simulink model "ElevatorPlant_Storage_A"  (R2015b)
(part 3 of 8)

      state Updating_button_0
        en:
        BUTTON=MAX_BUT;
      state Updating_button_1
        en:
        BUTTON=MIN_BUT;
      (junction 29277) -> Button_detection.Max_Min_assignment.Min_but [order 1] : [(MAX_BUT-FLOOR)>(FLOOR-MIN_BUT)]
      Button_detection.Max_Min_assignment.Min_but -> (junction 29278)
      (junction 29279) -> (junction 29277) [order 1] : [not(FLAG_STOP) && MOTION==2 && FLAG==3]
      (default) -> (junction 29279)
      (junction 29277) -> (junction 29280) [order 2]
      (junction 29278) -> (junction 29281)
      (junction 29279) -> (junction 29282) [order 2]
      (junction 29280) -> Button_detection.Max_Min_assignment.Max_but [order 1] : [(MAX_BUT-FLOOR)<(FLOOR-MIN_BUT)]
      Button_detection.Max_Min_assignment.Max_but -> (junction 29281)
      (junction 29280) -> Button_detection.Max_Min_assignment.First_but [order 2]
      (junction 29281) -> (junction 29284)
      Button_detection.Max_Min_assignment.First_but -> (junction 29283)
      (junction 29283) -> (junction 29282)
      (junction 29284) -> (junction 29283)
      (junction 29282) -> (junction 29285)
      (junction 29286) -> (junction 29287) [order 1] : [MOTION==0]
          | {MOTION=1;
          | UPDATE=true;}
      (junction 29287) -> Button_detection.Max_Min_assignment.Max_but1 [order 1] : [BUTTON_UP(2)]
      Button_detection.Max_Min_assignment.Max_but1 -> (junction 29288)
      (junction 29285) -> (junction 29286) [order 1] : [BUTTON==FLOOR && EXTEND]
          | {EXTEND=false;}
      (junction 29285) -> (junction 29299) [order 2]
      (junction 29286) -> (junction 29291) [order 2]
      (junction 29287) -> (junction 29289) [order 2]
      (junction 29288) -> (junction 29290)
      (junction 29289) -> Button_detection.Max_Min_assignment.Max_but2 [order 1] : [BUTTON_UP(1)]
      Button_detection.Max_Min_assignment.Max_but2 -> (junction 29290)
      (junction 29289) -> Button_detection.Max_Min_assignment.Max_but3 [order 2]
      (junction 29290) -> (junction 29293)
      Button_detection.Max_Min_assignment.Max_but3 -> (junction 29292)
      (junction 29292) -> (junction 29291)
      (junction 29293) -> (junction 29292)
      (junction 29291) -> (junction 29294)
      (junction 29294) -> (junction 29295) [order 1] : [MOTION==1]
          | {MOTION=0;
          | UPDATE=true;}
      (junction 29295) -> Button_detection.Max_Min_assignment.Min_but1 [order 1] : [BUTTON_DOWN(1)]
      Button_detection.Max_Min_assignment.Min_but1 -> (junction 29296)
      (junction 29294) -> (junction 29300) [order 2]
      (junction 29295) -> (junction 29297) [order 2]
      (junction 29296) -> (junction 29298)
      (junction 29297) -> Button_detection.Max_Min_assignment.Min_but2 [order 1] : [BUTTON_DOWN(2)]
      Button_detection.Max_Min_assignment.Min_but2 -> (junction 29298)
      (junction 29297) -> Button_detection.Max_Min_assignment.Min_but3 [order 2]
      (junction 29298) -> (junction 29302)
      Button_detection.Max_Min_assignment.Min_but3 -> (junction 29301)
      (junction 29300) -> (junction 29299)
      (junction 29301) -> (junction 29300)
      (junction 29302) -> (junction 29301)
      (junction 29299) -> (junction 29304)
      Button_detection.Max_Min_assignment.MAX -> (junction 29303)
      (junction 29304) -> (junction 29305) [order 1] : [PUSHED]
      (junction 29305) -> (junction 29306) [order 1] : [not(BUT_TEMP==FLOOR) || not(MOTION==2)]
      (junction 29306) -> Button_detection.Max_Min_assignment.MAX [order 1] : [MAX_BUT<BUT_TEMP && not(UPDATE)]
      (junction 29303) -> (junction 29308)
      (junction 29304) -> (junction 29318) [order 2]
      (junction 29305) -> (junction 29311) [order 2]
      (junction 29306) -> (junction 29307) [order 2]
      (junction 29308) -> (junction 29307)
      (junction 29307) -> (junction 29309)
      (junction 29309) -> Button_detection.Max_Min_assignment.MIN [order 1] : [MIN_BUT>BUT_TEMP && not(UPDATE)]
      Button_detection.Max_Min_assignment.MIN -> (junction 29310)
      (junction 29309) -> (junction 29312) [order 2]
      (junction 29310) -> (junction 29313)
      (junction 29312) -> (junction 29311)
      (junction 29313) -> (junction 29312)
      (junction 29311) -> (junction 29314)
      (junction 29314) -> Button_detection.Max_Min_assignment.Updating_button_0 [order 1] : [MOTION==0]
      Button_detection.Max_Min_assignment.Updating_button_0 -> (junction 29315)
      (junction 29314) -> (junction 29316) [order 2]
      (junction 29315) -> (junction 29317)
      (junction 29316) -> Button_detection.Max_Min_assignment.Updating_button_1 [order 1] : [MOTION==1]
      Button_detection.Max_Min_assignment.Updating_button_1 -> (junction 29317)
      (junction 29316) -> (junction 29319) [order 2]
      (junction 29317) -> (junction 29320)
      (junction 29319) -> (junction 29318)
      (junction 29320) -> (junction 29319)
    state GoTo_PositionControl
      en:
      BUTTON=BUT_TEMP;
      FLAG=2;
    state Emergency
      en:
      FLAG_EMG=true;
      FLAG=4;
    state Timer_EME
      state Set_tmr
        en:
        Q_EME=true;
      state Counting
        en:
        ET_EME= ET_EME + 1;
        Q_EME=false;
      state Set
        en:
        IN_EME=true;
        PT_EME=3;
      (junction 29410) -> Button_detection.Timer_EME.Set_tmr [order 1] : [ET_EME==PT_EME]
      Button_detection.Timer_EME.Set_tmr -> (junction 29411)
      Button_detection.Timer_EME.Counting -> (junction 29410)
      (junction 29410) -> (junction 29411) [order 2]
      (default) -> Button_detection.Timer_EME.Set
      Button_detection.Timer_EME.Set -> (junction 29412)
      (junction 29412) -> Button_detection.Timer_EME.Counting [order 1] : [ET_EME<PT_EME]
      (junction 29412) -> (junction 29411) [order 2]
    state Not_Emergency
      en:
      IN_EME=false;
      ET_EME=0;
    state SwitchingOFF_LEDs
      en:
      LPD3=false;
      LPD2=false;
      LPS2=false;
      LPD1=false;
      LPS1=false;
      LPS0=false;
    (default) -> (junction 29011)
    (junction 29011) -> (junction 29012) [order 1] : [FLAG==1 && not(PUSHED)]
        | {BUTTON=FLOOR;
        | BUT_TEMP=BUTTON;
        | BUT_1=FLOOR;}
    (junction 29012) -> Button_detection.Timer_LL [order 1] : [not(FLAG_STOP)]
    Button_detection.Save_energy -> (junction 29013)
    Button_detection.Timer_LL -> Button_detection.Save_energy
    (junction 29012) -> (junction 29015) [order 2]
    (junction 29011) -> (junction 29014) [order 2]
    (junction 29013) -> (junction 29016)
    (junction 29015) -> (junction 29014)
    (junction 29016) -> (junction 29015)
    (junction 29014) -> Button_detection.BUTTON_CAR
    Button_detection.BUTTON_UP -> Button_detection.BUTTON_DOWN
    Button_detection.BUTTON_DOWN -> Button_detection.Max_Min_assignment
    Button_detection.Max_Min_assignment -> (junction 29017)
    Button_detection.BUTTON_CAR -> Button_detection.BUTTON_UP
    (junction 29017) -> (junction 29019)
    (junction 29019) -> (junction 29018)
    (junction 29018) -> (junction 29021)
    Button_detection.GoTo_PositionControl -> (junction 29020)
    (junction 29021) -> (junction 29022) [order 1] : [FLAG==1]
    (junction 29022) -> Button_detection.GoTo_PositionControl [order 1] : [PUSHED]
    (junction 29020) -> (junction 29024)
    (junction 29021) -> (junction 29032) [order 2]
    (junction 29022) -> (junction 29023) [order 2]
    (junction 29024) -> (junction 29023)
    (junction 29023) -> (junction 29026)
    Button_detection.Emergency -> (junction 29025)
    (junction 29026) -> Button_detection.Timer_EME [order 1] : [STOP]
        | {IN_LL=false; ET_LL=0;FLAG=1;}
    Button_detection.Timer_EME -> (junction 29027)
    (junction 29027) -> Button_detection.Emergency [order 1] : [Q_EME]
    (junction 29025) -> (junction 29029)
    (junction 29026) -> Button_detection.Not_Emergency [order 2]
    (junction 29027) -> (junction 29028) [order 2]
    (junction 29029) -> (junction 29028)
    (junction 29028) -> (junction 29031)
    Button_detection.Not_Emergency -> (junction 29031)
    Button_detection.SwitchingOFF_LEDs -> (junction 29030)
    (junction 29031) -> Button_detection.SwitchingOFF_LEDs [order 1] : [FLAG_STOP && FLAG==2]
    (junction 29030) -> (junction 29034)
    (junction 29031) -> (junction 29033) [order 2]
    (junction 29033) -> (junction 29032)
    (junction 29034) -> (junction 29033)
  state Position_control
    state Going_UP
      en:
      SALI=true;
      MOTION=0;
      FLAG_STOP=false;
    state Button_detection
      state Save_energy
        en:
        LL=not(Q_LL);
      state Timer_LL
        state Set_tmr
          en:
          Q_LL=true;
        state Counting
          en:
          ET_LL= ET_LL + 1;
          Q_LL=false;
        state Set
          en:
          IN_LL=true;
          PT_LL=10;
        (junction 68131) -> Position_control.Button_detection.Timer_LL.Set_tmr [order 1] : [ET_LL==PT_LL]
        Position_control.Button_detection.Timer_LL.Set_tmr -> (junction 68132)
        Position_control.Button_detection.Timer_LL.Counting -> (junction 68131)
        (junction 68131) -> (junction 68132) [order 2]
        (default) -> Position_control.Button_detection.Timer_LL.Set
        Position_control.Button_detection.Timer_LL.Set -> (junction 68133)
        (junction 68133) -> Position_control.Button_detection.Timer_LL.Counting [order 1] : [ET_LL<PT_LL]
        (junction 68133) -> (junction 68132) [order 2]
      state BUTTON_DOWN
        state Button_DOWN_1
          en:
          BUTTON_DOWN(2)=true;
          BUT_TEMP=1;
          LPD1=true;
          PUSHED=true;
          UPDATE=false;
          IN_LL=false; ET_LL=0;
        state First_but_1
          en:
          BUT_1=BUT_TEMP;
          FIRST_BUT=false;
        state Button_DOWN_2
          en:
          BUTTON_DOWN(3)=true;
          BUT_TEMP=2;
          LPD2=true;
          PUSHED=true;
          UPDATE=false;
          IN_LL=false; ET_LL=0;
        state First_but_2
          en:
          BUT_1=BUT_TEMP;
          FIRST_BUT=false;
        state Button_DOWN_3
          en:
          BUTTON_DOWN(4)=true;
          BUT_TEMP=3;
          LPD3=true;
          PUSHED=true;
          UPDATE=false;
          IN_LL=false; ET_LL=0;
        state First_but_3
          en:
          BUT_1=BUT_TEMP;
          FIRST_BUT=false;
        (default) -> (junction 68146)
        (junction 68146) -> Position_control.Button_detection.BUTTON_DOWN.Button_DOWN_1 [order 1] : [PD1]
        Position_control.Button_detection.BUTTON_DOWN.Button_DOWN_1 -> (junction 68147)
        (junction 68147) -> Position_control.Button_detection.BUTTON_DOWN.First_but_1 [order 1] : [FIRST_BUT && not(RPC1)]
        Position_control.Button_detection.BUTTON_DOWN.First_but_1 -> (junction 68148)
        (junction 68146) -> (junction 68149) [order 2]
        (junction 68147) -> (junction 68150) [order 2]
        (junction 68148) -> (junction 68151)
        (junction 68150) -> (junction 68149)
        (junction 68151) -> (junction 68150)
        (junction 68149) -> (junction 68152)
        (junction 68152) -> Position_control.Button_detection.BUTTON_DOWN.Button_DOWN_2 [order 1] : [PD2]
        Position_control.Button_detection.BUTTON_DOWN.Button_DOWN_2 -> (junction 68153)
        (junction 68153) -> Position_control.Button_detection.BUTTON_DOWN.First_but_2 [order 1] : [FIRST_BUT && not(RPC2)]
        Position_control.Button_detection.BUTTON_DOWN.First_but_2 -> (junction 68154)
        (junction 68152) -> (junction 68155) [order 2]
        (junction 68153) -> (junction 68156) [order 2]
        (junction 68154) -> (junction 68157)
        (junction 68156) -> (junction 68155)
        (junction 68157) -> (junction 68156)
        (junction 68155) -> (junction 68158)
        (junction 68158) -> Position_control.Button_detection.BUTTON_DOWN.Button_DOWN_3 [order 1] : [PD3]
        Position_control.Button_detection.BUTTON_DOWN.Button_DOWN_3 -> (junction 68159)
        (junction 68159) -> Position_control.Button_detection.BUTTON_DOWN.First_but_3 [order 1] : [FIRST_BUT && not(RPC3)]
        Position_control.Button_detection.BUTTON_DOWN.First_but_3 -> (junction 68160)
        (junction 68158) -> (junction 68161) [order 2]
        (junction 68159) -> (junction 68162) [order 2]
        (junction 68160) -> (junction 68163)
        (junction 68162) -> (junction 68161)
        (junction 68163) -> (junction 68162)
      state BUTTON_CAR
        state Button_CAR_0
          en:
          BUTTON_CAR(1)=true;
          BUT_TEMP=0;
          LPC0=true;
          PUSHED=true;
          UPDATE=false;
          IN_LL=false; ET_LL=0;
        state First_but_0
          en:
          BUT_1=BUT_TEMP;
          FIRST_BUT=false;
        state Button_CAR_1
          en:
          BUTTON_CAR(2)=true;
          BUT_TEMP=1;
          LPC1=true;
          PUSHED=true;
          UPDATE=false;
          IN_LL=false; ET_LL=0;
        state First_but_1
          en:
          BUT_1=BUT_TEMP;
          FIRST_BUT=false;
        state Button_CAR_2
          en:
          BUTTON_CAR(3)=true;
          BUT_TEMP=2;
          LPC2=true;
          PUSHED=true;
          UPDATE=false;
          IN_LL=false; ET_LL=0;
        state First_but_2
          en:
          BUT_1=BUT_TEMP;
          FIRST_BUT=false;
        state Button_CAR_3
          en:
          BUTTON_CAR(4)=true;
          BUT_TEMP=3;
          LPC3=true;
          PUSHED=true;
          UPDATE=false;
          IN_LL=false; ET_LL=0;
        state First_but_3
          en:
          BUT_1=BUT_TEMP;
          FIRST_BUT=false;
        (default) -> (junction 68201)
        (junction 68201) -> Position_control.Button_detection.BUTTON_CAR.Button_CAR_0 [order 1] : [P0]
        Position_control.Button_detection.BUTTON_CAR.Button_CAR_0 -> (junction 68202)
        (junction 68202) -> Position_control.Button_detection.BUTTON_CAR.First_but_0 [order 1] : [FIRST_BUT && not(RPC0)]
        Position_control.Button_detection.BUTTON_CAR.First_but_0 -> (junction 68203)
        (junction 68201) -> (junction 68204) [order 2]
        (junction 68202) -> (junction 68205) [order 2]
        (junction 68203) -> (junction 68206)
        (junction 68205) -> (junction 68204)
        (junction 68206) -> (junction 68205)
        (junction 68204) -> (junction 68209)
        Position_control.Button_detection.BUTTON_CAR.Button_CAR_1 -> (junction 68207)
        (junction 68207) -> Position_control.Button_detection.BUTTON_CAR.First_but_1 [order 1] : [FIRST_BUT && not(RPC1)]
        Position_control.Button_detection.BUTTON_CAR.First_but_1 -> (junction 68208)
        (junction 68207) -> (junction 68211) [order 2]
        (junction 68208) -> (junction 68212)
        (junction 68209) -> Position_control.Button_detection.BUTTON_CAR.Button_CAR_1 [order 1] : [P1]
        (junction 68209) -> (junction 68210) [order 2]
        (junction 68211) -> (junction 68210)
        (junction 68212) -> (junction 68211)
        (junction 68210) -> (junction 68213)
        (junction 68213) -> Position_control.Button_detection.BUTTON_CAR.Button_CAR_2 [order 1] : [P2]
        Position_control.Button_detection.BUTTON_CAR.Button_CAR_2 -> (junction 68214)
        (junction 68214) -> Position_control.Button_detection.BUTTON_CAR.First_but_2 [order 1] : [FIRST_BUT && not(RPC2)]
        Position_control.Button_detection.BUTTON_CAR.First_but_2 -> (junction 68215)
        (junction 68213) -> (junction 68216) [order 2]
        (junction 68214) -> (junction 68217) [order 2]
        (junction 68215) -> (junction 68218)
        (junction 68217) -> (junction 68216)
        (junction 68218) -> (junction 68217)
        (junction 68216) -> (junction 68219)
        (junction 68219) -> Position_control.Button_detection.BUTTON_CAR.Button_CAR_3 [order 1] : [P3]
        Position_control.Button_detection.BUTTON_CAR.Button_CAR_3 -> (junction 68220)
        (junction 68220) -> Position_control.Button_detection.BUTTON_CAR.First_but_3 [order 1] : [FIRST_BUT && not(RPC3)]
        Position_control.Button_detection.BUTTON_CAR.First_but_3 -> (junction 68221)
        (junction 68219) -> (junction 68222) [order 2]
        (junction 68220) -> (junction 68223) [order 2]
        (junction 68221) -> (junction 68224)
        (junction 68223) -> (junction 68222)
        (junction 68224) -> (junction 68223)
      state BUTTON_UP
        state Button_UP_0
          en:
          BUTTON_UP(1)=true;
          BUT_TEMP=0;
          LPS0=true;
          PUSHED=true;
          UPDATE=false;
          IN_LL=false; ET_LL=0;
        state First_but_0
          en:
          BUT_1=BUT_TEMP;
          FIRST_BUT=false;
        state Button_UP_1
          en:
          BUTTON_UP(2)=true;
          BUT_TEMP=1;
          LPS1=true;
          PUSHED=true;
          UPDATE=false;
          IN_LL=false; ET_LL=0;
        state First_but_1
          en:
          BUT_1=BUT_TEMP;
          FIRST_BUT=false;
        state Button_UP_2
          en:
          BUTTON_UP(3)=true;
          BUT_TEMP=2;
          LPS2=true;
          PUSHED=true;
          UPDATE=false;
          IN_LL=false; ET_LL=0;
        state First_but_2
          en:
          BUT_1=BUT_TEMP;
          FIRST_BUT=false;
        (junction 68274) -> Position_control.Button_detection.BUTTON_UP.Button_UP_0 [order 1] : [PS0]
        Position_control.Button_detection.BUTTON_UP.Button_UP_0 -> (junction 68275)
        (junction 68275) -> Position_control.Button_detection.BUTTON_UP.First_but_0 [order 1] : [FIRST_BUT && not(RPC0)]
        Position_control.Button_detection.BUTTON_UP.First_but_0 -> (junction 68276)
        (default) -> (junction 68274)
        (junction 68274) -> (junction 68279) [order 2]
        (junction 68275) -> (junction 68277) [order 2]
        (junction 68276) -> (junction 68278)
        (junction 68278) -> (junction 68277)
        (junction 68277) -> (junction 68279)
        (junction 68279) -> (junction 68280)
        (junction 68280) -> Position_control.Button_detection.BUTTON_UP.Button_UP_1 [order 1] : [PS1]
        Position_control.Button_detection.BUTTON_UP.Button_UP_1 -> (junction 68281)
        (junction 68281) -> Position_control.Button_detection.BUTTON_UP.First_but_1 [order 1] : [FIRST_BUT && not(RPC1)]
        Position_control.Button_detection.BUTTON_UP.First_but_1 -> (junction 68282)
        (junction 68280) -> (junction 68283) [order 2]
        (junction 68281) -> (junction 68284) [order 2]
        (junction 68282) -> (junction 68285)
        (junction 68284) -> (junction 68283)
        (junction 68285) -> (junction 68284)
        (junction 68283) -> (junction 68287)
        Position_control.Button_detection.BUTTON_UP.First_but_2 -> (junction 68286)
        (junction 68286) -> (junction 68291)
        (junction 68287) -> Position_control.Button_detection.BUTTON_UP.Button_UP_2 [order 1] : [PS2]
        Position_control.Button_detection.BUTTON_UP.Button_UP_2 -> (junction 68288)
        (junction 68288) -> Position_control.Button_detection.BUTTON_UP.First_but_2 [order 1] : [FIRST_BUT && not(RPC2)]
        (junction 68287) -> (junction 68289) [order 2]
        (junction 68288) -> (junction 68290) [order 2]
        (junction 68290) -> (junction 68289)
        (junction 68291) -> (junction 68290)
      state Max_Min_assignment
        state Min_but
          en:
          BUTTON=MIN_BUT;
        state Max_but
          en:
          BUTTON=MAX_BUT;
        state First_but
          en:
          BUTTON=BUT_1;
        state Max_but1
          en:
          MAX_BUT=2;
        state Max_but2
          en:
          MAX_BUT=1;
        state Max_but3
          en:
          MAX_BUT=0;
        state Min_but1
          en:
          MIN_BUT=1;
        state Min_but2
          en:
          MIN_BUT=2;
        state Min_but3
          en:
          MIN_BUT=3;
        state MAX
          en:
          MAX_BUT=BUT_TEMP;
        state MIN
          en:
          MIN_BUT=BUT_TEMP;
        state Updating_button_0
          en:
          BUTTON=MAX_BUT;
        state Updating_button_1
          en:
          BUTTON=MIN_BUT;
        (junction 68329) -> Position_control.Button_detection.Max_Min_assignment.Min_but [order 1] : [(MAX_BUT-FLOOR)>(FLOOR-MIN_BUT)]
        Position_control.Button_detection.Max_Min_assignment.Min_but -> (junction 68330)
        (junction 68331) -> (junction 68329) [order 1] : [not(FLAG_STOP) && MOTION==2 && FLAG==3]
        (default) -> (junction 68331)
        (junction 68329) -> (junction 68332) [order 2]
        (junction 68330) -> (junction 68333)
        (junction 68331) -> (junction 68334) [order 2]
        (junction 68332) -> Position_control.Button_detection.Max_Min_assignment.Max_but [order 1] : [(MAX_BUT-FLOOR)<(FLOOR-MIN_BUT)]
        Position_control.Button_detection.Max_Min_assignment.Max_but -> (junction 68333)
        (junction 68332) -> Position_control.Button_detection.Max_Min_assignment.First_but [order 2]
        (junction 68333) -> (junction 68336)
        Position_control.Button_detection.Max_Min_assignment.First_but -> (junction 68335)
        (junction 68335) -> (junction 68334)
        (junction 68336) -> (junction 68335)
        (junction 68334) -> (junction 68337)
        (junction 68338) -> (junction 68339) [order 1] : [MOTION==0]
            | {MOTION=1;
            | UPDATE=true;}
        (junction 68339) -> Position_control.Button_detection.Max_Min_assignment.Max_but1 [order 1] : [BUTTON_UP(2)]
        Position_control.Button_detection.Max_Min_assignment.Max_but1 -> (junction 68340)
        (junction 68337) -> (junction 68338) [order 1] : [BUTTON==FLOOR && EXTEND]
            | {EXTEND=false;}
        (junction 68337) -> (junction 68351) [order 2]
        (junction 68338) -> (junction 68343) [order 2]
        (junction 68339) -> (junction 68341) [order 2]
        (junction 68340) -> (junction 68342)
        (junction 68341) -> Position_control.Button_detection.Max_Min_assignment.Max_but2 [order 1] : [BUTTON_UP(1)]
        Position_control.Button_detection.Max_Min_assignment.Max_but2 -> (junction 68342)
        (junction 68341) -> Position_control.Button_detection.Max_Min_assignment.Max_but3 [order 2]
        (junction 68342) -> (junction 68345)
        Position_control.Button_detection.Max_Min_assignment.Max_but3 -> (junction 68344)
        (junction 68344) -> (junction 68343)
        (junction 68345) -> (junction 68344)
        (junction 68343) -> (junction 68346)
        (junction 68346) -> (junction 68347) [order 1] : [MOTION==1]
            | {MOTION=0;
            | UPDATE=true;}
        (junction 68347) -> Position_control.Button_detection.Max_Min_assignment.Min_but1 [order 1] : [BUTTON_DOWN(1)]
        Position_control.Button_detection.Max_Min_assignment.Min_but1 -> (junction 68348)
        (junction 68346) -> (junction 68352) [order 2]
        (junction 68347) -> (junction 68349) [order 2]
        (junction 68348) -> (junction 68350)
        (junction 68349) -> Position_control.Button_detection.Max_Min_assignment.Min_but2 [order 1] : [BUTTON_DOWN(2)]
        Position_control.Button_detection.Max_Min_assignment.Min_but2 -> (junction 68350)
        (junction 68349) -> Position_control.Button_detection.Max_Min_assignment.Min_but3 [order 2]
        (junction 68350) -> (junction 68354)
        Position_control.Button_detection.Max_Min_assignment.Min_but3 -> (junction 68353)
        (junction 68352) -> (junction 68351)
        (junction 68353) -> (junction 68352)
        (junction 68354) -> (junction 68353)
        (junction 68351) -> (junction 68356)
        Position_control.Button_detection.Max_Min_assignment.MAX -> (junction 68355)
        (junction 68356) -> (junction 68357) [order 1] : [PUSHED]
        (junction 68357) -> (junction 68358) [order 1] : [not(BUT_TEMP==FLOOR) || not(MOTION==2)]
        (junction 68358) -> Position_control.Button_detection.Max_Min_assignment.MAX [order 1] : [MAX_BUT<BUT_TEMP && not(UPDATE)]
        (junction 68355) -> (junction 68360)
        (junction 68356) -> (junction 68370) [order 2]
        (junction 68357) -> (junction 68363) [order 2]
        (junction 68358) -> (junction 68359) [order 2]
        (junction 68360) -> (junction 68359)
        (junction 68359) -> (junction 68361)
        (junction 68361) -> Position_control.Button_detection.Max_Min_assignment.MIN [order 1] : [MIN_BUT>BUT_TEMP && not(UPDATE)]
        Position_control.Button_detection.Max_Min_assignment.MIN -> (junction 68362)
        (junction 68361) -> (junction 68364) [order 2]
        (junction 68362) -> (junction 68365)
        (junction 68364) -> (junction 68363)
        (junction 68365) -> (junction 68364)
        (junction 68363) -> (junction 68366)
        (junction 68366) -> Position_control.Button_detection.Max_Min_assignment.Updating_button_0 [order 1] : [MOTION==0]
        Position_control.Button_detection.Max_Min_assignment.Updating_button_0 -> (junction 68367)
        (junction 68366) -> (junction 68368) [order 2]
        (junction 68367) -> (junction 68369)
        (junction 68368) -> Position_control.Button_detection.Max_Min_assignment.Updating_button_1 [order 1] : [MOTION==1]
        Position_control.Button_detection.Max_Min_assignment.Updating_button_1 -> (junction 68369)
        (junction 68368) -> (junction 68371) [order 2]
        (junction 68369) -> (junction 68372)
        (junction 68371) -> (junction 68370)
        (junction 68372) -> (junction 68371)
      state GoTo_PositionControl
        en:
        BUTTON=BUT_TEMP;
        FLAG=2;
      state Emergency
        en:
        FLAG_EMG=true;
        FLAG=4;
      state Timer_EME
        state Set_tmr
          en:
          Q_EME=true;
        state Counting
          en:
          ET_EME= ET_EME + 1;
          Q_EME=false;
        state Set
          en:
          IN_EME=true;
          PT_EME=3;
        (junction 68462) -> Position_control.Button_detection.Timer_EME.Set_tmr [order 1] : [ET_EME==PT_EME]
        Position_control.Button_detection.Timer_EME.Set_tmr -> (junction 68463)
        Position_control.Button_detection.Timer_EME.Counting -> (junction 68462)
        (junction 68462) -> (junction 68463) [order 2]
        (default) -> Position_control.Button_detection.Timer_EME.Set
        Position_control.Button_detection.Timer_EME.Set -> (junction 68464)
        (junction 68464) -> Position_control.Button_detection.Timer_EME.Counting [order 1] : [ET_EME<PT_EME]
        (junction 68464) -> (junction 68463) [order 2]
      state Not_Emergency
        en:
        IN_EME=false;
        ET_EME=0;
      state SwitchingOFF_LEDs
        en:
        LPD3=false;
        LPD2=false;
        LPS2=false;
        LPD1=false;
        LPS1=false;
        LPS0=false;
      (default) -> (junction 68063)
      (junction 68063) -> (junction 68064) [order 1] : [FLAG==1 && not(PUSHED)]
          | {BUTTON=FLOOR;
          | BUT_TEMP=BUTTON;
          | BUT_1=FLOOR;}
      (junction 68064) -> Position_control.Button_detection.Timer_LL [order 1] : [not(FLAG_STOP)]
      Position_control.Button_detection.Save_energy -> (junction 68065)
      Position_control.Button_detection.Timer_LL -> Position_control.Button_detection.Save_energy
      (junction 68064) -> (junction 68067) [order 2]
      (junction 68063) -> (junction 68066) [order 2]
      (junction 68065) -> (junction 68068)
      (junction 68067) -> (junction 68066)
      (junction 68068) -> (junction 68067)
      (junction 68066) -> Position_control.Button_detection.BUTTON_CAR
      Position_control.Button_detection.BUTTON_UP -> Position_control.Button_detection.BUTTON_DOWN
      Position_control.Button_detection.BUTTON_DOWN -> Position_control.Button_detection.Max_Min_assignment
      Position_control.Button_detection.Max_Min_assignment -> (junction 68069)
      Position_control.Button_detection.BUTTON_CAR -> Position_control.Button_detection.BUTTON_UP
      (junction 68069) -> (junction 68071)
      (junction 68071) -> (junction 68070)
      (junction 68070) -> (junction 68073)
      Position_control.Button_detection.GoTo_PositionControl -> (junction 68072)
      (junction 68073) -> (junction 68074) [order 1] : [FLAG==1]
      (junction 68074) -> Position_control.Button_detection.GoTo_PositionControl [order 1] : [PUSHED]
      (junction 68072) -> (junction 68076)
      (junction 68073) -> (junction 68084) [order 2]
      (junction 68074) -> (junction 68075) [order 2]
      (junction 68076) -> (junction 68075)
      (junction 68075) -> (junction 68078)
      Position_control.Button_detection.Emergency -> (junction 68077)
      (junction 68078) -> Position_control.Button_detection.Timer_EME [order 1] : [STOP]
          | {IN_LL=false; ET_LL=0;FLAG=1;}
      Position_control.Button_detection.Timer_EME -> (junction 68079)
      (junction 68079) -> Position_control.Button_detection.Emergency [order 1] : [Q_EME]
      (junction 68077) -> (junction 68081)
      (junction 68078) -> Position_control.Button_detection.Not_Emergency [order 2]
      (junction 68079) -> (junction 68080) [order 2]
      (junction 68081) -> (junction 68080)
      (junction 68080) -> (junction 68083)
      Position_control.Button_detection.Not_Emergency -> (junction 68083)
      Position_control.Button_detection.SwitchingOFF_LEDs -> (junction 68082)
      (junction 68083) -> Position_control.Button_detection.SwitchingOFF_LEDs [order 1] : [FLAG_STOP && FLAG==2]
      (junction 68082) -> (junction 68086)
      (junction 68083) -> (junction 68085) [order 2]
      (junction 68085) -> (junction 68084)
      (junction 68086) -> (junction 68085)
    state INT_Stop
      state Stop
        en: SALI=false;
        FLAG=3;
      state Stop1
        en: SALI=false;
        FLAG=3;
      state Stop2
        en: SCENDI=false;
        FLAG=3;
      state Stop3
        en: SCENDI=false;
        FLAG=3;
      Position_control.INT_Stop.Stop -> (junction 29850)
      (default) -> (junction 12494)
      (junction 12494) -> (junction 12497) [order 1] : [MOTION==0]
      (junction 12497) -> (junction 12481) [order 1] : [FLOOR==1]
      (junction 12481) -> Position_control.INT_Stop.Stop [order 1] : [RPC1 && (BUTTON_CAR(2) || BUTTON_UP(2))]
      (junction 29850) -> (junction 29857)
      (junction 12494) -> (junction 29876) [order 2]
      (junction 12497) -> (junction 29848) [order 2]
      (junction 12481) -> (junction 29855) [order 2]
      (junction 29855) -> (junction 29857)
      (junction 29857) -> (junction 29852)
      (junction 12487) -> Position_control.INT_Stop.Stop1 [order 1] : [RPC2 && (BUTTON_CAR(3) || BUTTON_UP(3))]
      (junction 29848) -> (junction 12487) [order 1] : [FLOOR==2]
      Position_control.INT_Stop.Stop1 -> (junction 29852)
      (junction 29848) -> (junction 29874) [order 2]
      (junction 12487) -> (junction 29861) [order 2]
      (junction 29852) -> (junction 29862)
      (junction 29861) -> (junction 29862)
      (junction 29862) -> (junction 29866)
      (junction 29874) -> (junction 29876)
      (junction 29866) -> (junction 29874)
      (junction 29876) -> (junction 29878)
      Position_control.INT_Stop.Stop2 -> (junction 29880)
      (junction 12488) -> Position_control.INT_Stop.Stop2 [order 1] : [RPC1 && (BUTTON_CAR(2) || BUTTON_DOWN(2))]
      (junction 29878) -> (junction 12489) [order 1] : [MOTION==1]
      (junction 12489) -> (junction 12488) [order 1] : [FLOOR==1]
      (junction 29880) -> (junction 29882)
      (junction 29878) -> (junction 29902) [order 2]
      (junction 12489) -> (junction 29888) [order 2]
      (junction 12488) -> (junction 29883) [order 2]
      (junction 29883) -> (junction 29882)
      Position_control.INT_Stop.Stop3 -> (junction 29890)
      (junction 29888) -> (junction 12498) [order 1] : [FLOOR==2]
      (junction 12498) -> Position_control.INT_Stop.Stop3 [order 1] : [RPC2 && (BUTTON_CAR(3) || BUTTON_DOWN(3))]
      (junction 29890) -> (junction 29892)
      (junction 29888) -> (junction 29899) [order 2]
      (junction 12498) -> (junction 29893) [order 2]
      (junction 29893) -> (junction 29892)
      (junction 29892) -> (junction 29897)
      (junction 29899) -> (junction 29902)
      (junction 29897) -> (junction 29899)
    state Going_DOWN
      en:
      SCENDI=true;
      MOTION=1;
      FLAG_STOP=false;
    state INT_Stop1
      state Stop
        en: SALI=false;
        FLAG=3;
      state Stop1
        en: SALI=false;
        FLAG=3;
      state Stop2
        en: SCENDI=false;
        FLAG=3;
      state Stop3
        en: SCENDI=false;
        FLAG=3;
      Position_control.INT_Stop1.Stop -> (junction 29906)
      (default) -> (junction 29907)
      (junction 29907) -> (junction 29908) [order 1] : [MOTION==0]
      (junction 29908) -> (junction 29909) [order 1] : [FLOOR==1]
      (junction 29909) -> Position_control.INT_Stop1.Stop [order 1] : [RPC1 && (BUTTON_CAR(2) || BUTTON_UP(2))]
      (junction 29906) -> (junction 29911)
      (junction 29907) -> (junction 29917) [order 2]
      (junction 29908) -> (junction 29912) [order 2]
      (junction 29909) -> (junction 29910) [order 2]
      (junction 29910) -> (junction 29911)
      (junction 29911) -> (junction 29914)
      (junction 29913) -> Position_control.INT_Stop1.Stop1 [order 1] : [RPC2 && (BUTTON_CAR(3) || BUTTON_UP(3))]
      (junction 29912) -> (junction 29913) [order 1] : [FLOOR==2]
      Position_control.INT_Stop1.Stop1 -> (junction 29914)
      (junction 29912) -> (junction 29918) [order 2]
      (junction 29913) -> (junction 29915) [order 2]
      (junction 29914) -> (junction 29916)
      (junction 29915) -> (junction 29916)
      (junction 29916) -> (junction 29919)
      (junction 29918) -> (junction 29917)
      (junction 29919) -> (junction 29918)
      (junction 29917) -> (junction 29921)
      Position_control.INT_Stop1.Stop2 -> (junction 29920)
      (junction 29923) -> Position_control.INT_Stop1.Stop2 [order 1] : [RPC1 && (BUTTON_CAR(2) || BUTTON_DOWN(2))]
      (junction 29921) -> (junction 29922) [order 1] : [MOTION==1]
      (junction 29922) -> (junction 29923) [order 1] : [FLOOR==1]
      (junction 29920) -> (junction 29925)
      (junction 29921) -> (junction 29931) [order 2]
      (junction 29922) -> (junction 29927) [order 2]
      (junction 29923) -> (junction 29924) [order 2]
      (junction 29924) -> (junction 29925)
      Position_control.INT_Stop1.Stop3 -> (junction 29926)
      (junction 29927) -> (junction 29928) [order 1] : [FLOOR==2]
      (junction 29928) -> Position_control.INT_Stop1.Stop3 [order 1] : [RPC2 && (BUTTON_CAR(3) || BUTTON_DOWN(3))]
      (junction 29926) -> (junction 29930)
      (junction 29927) -> (junction 29932) [order 2]
      (junction 29928) -> (junction 29929) [order 2]
      (junction 29929) -> (junction 29930)
      (junction 29930) -> (junction 29933)
      (junction 29932) -> (junction 29931)
      (junction 29933) -> (junction 29932)
    state AFTER_STOP
      state Return_DOWN
        en:
        SCENDI=true;
      state Return_UP
        en:
        SALI=true;
        MOTION=0;
      (default) -> (junction 58122)
      (junction 58122) -> (junction 58123) [order 1] : [MOTION_TEMP==0]
      (junction 58123) -> Return_DOWN [order 1] : [not(( RPC0 && BUTTON==0 ) || ( RPC1 && BUTTON==1 ) || ( RPC2 && BUTTON==2 ) || ( RPC3 && BUTTON==3 ) || (STOP))]
      Return_DOWN -> (junction 58124)
      (junction 58122) -> (junction 58116) [order 2]
      (junction 58123) -> (junction 58111) [order 2] : {FLAG_STOP=false;}
      (junction 58124) -> (junction 58126)
      (junction 58111) -> (junction 58126)
      (junction 58126) -> (junction 58128)
      (junction 58116) -> (junction 58127) [order 1] : [MOTION_TEMP==1]
      (junction 58127) -> Return_UP [order 1] : [not(( RPC0 && BUTTON==0 ) || ( RPC1 && BUTTON==1 ) || ( RPC2 && BUTTON==2 ) || ( RPC3 && BUTTON==3 ) || (STOP))]
      Return_UP -> (junction 58128)
      (junction 58116) -> (junction 58117) [order 2]
      (junction 58127) -> (junction 58112) [order 2] : {FLAG_STOP=false;}
      (junction 58128) -> (junction 58115)
      (junction 58112) -> (junction 58115)
      (junction 58115) -> (junction 58120)
      (junction 58117) -> (junction 58120)
    state TARGET_REACHED
      en:
      FLAG=3;
    state STOP
      en:
      MAX_BUT=0;
      MIN_BUT=3;
      FLAG=1;
      BUTTON_CAR(1)=false;
      BUTTON_CAR(2)=false;
      BUTTON_CAR(3)=false;
      BUTTON_CAR(4)=false;
      BUTTON_UP(1)=false;
      BUTTON_UP(2)=false;
      BUTTON_UP(3)=false;
      BUTTON_UP(4)=false;
      BUTTON_DOWN(1)=false;
      BUTTON_DOWN(2)=false;
      BUTTON_DOWN(3)=false;
      BUTTON_DOWN(4)=false;
      PUSHED=false;
      LPD3=true;
      LPD2=true;
      LPS2=true;
      LPD1=true;
      LPS1=true;
      LPS0=true;
      FLAG_STOP=true;
      BUTTON=FLOOR;
      FIRST_BUT=true;
      MOTION=2;
    state Motion_Updating
      en:
      MOTION_TEMP=MOTION;
    (default) -> Position_control.Button_detection
    Position_control.Button_detection -> (junction 12336)
    (junction 12336) -> Going_UP [order 1] : [BUTTON>FLOOR && not(STOP)]
    INT_Stop -> (junction 30004)
    Going_UP -> INT_Stop
    (junction 12336) -> (junction 29842) [order 2]
    (junction 30004) -> (junction 29846)
    (junction 29842) -> Going_DOWN [order 1] : [BUTTON<FLOOR && not(STOP)]
    INT_Stop1 -> (junction 29846)
    Going_DOWN -> INT_Stop1
    (junction 29842) -> (junction 29981) [order 2]
    (junction 29846) -> (junction 30014)
    (junction 29981) -> AFTER_STOP [order 1] : [BUTTON==FLOOR && FLAG_STOP]
    AFTER_STOP -> (junction 30014)
    (junction 29981) -> (junction 12332) [order 2] : {SALI=false; SCENDI=false;}
    (junction 30014) -> (junction 30011)
    (junction 12332) -> TARGET_REACHED [order 1] : [RPC0 || RPC1 || RPC2 || RPC3]
    TARGET_REACHED -> (junction 30024)
    (junction 30024) -> (junction 30011)
    (junction 12332) -> STOP [order 2]
    (junction 30008) -> (junction 30024)
    STOP -> Motion_Updating : [MOTION==0 || MOTION==1]
    Motion_Updating -> (junction 30008)
  state OpCl_doors
    state OpCl_0
      state Closing0
        state Reset
          state Reset_0
            en:
            LPS0=false;
            BUTTON_CAR(1)=false;
            BUTTON_UP(1)=false;
          state Reset_1
            en:
            LPS1=false;
            LPD1=false;
            BUTTON_CAR(2)=false;
            BUTTON_UP(2)=false;
            BUTTON_DOWN(2)=false;
          state Reset_2
            en:
            LPS2=false;
            LPD2=false;
            BUTTON_CAR(3)=false;
            BUTTON_UP(3)=false;
            BUTTON_DOWN(3)=false;
          state Reset_3
            en:
            LPD3=false;
            BUTTON_CAR(4)=false;
            BUTTON_DOWN(4)=false;
          (default) -> (junction 68935)
          (junction 68935) -> OpCl_doors.OpCl_0.Closing0.Reset.Reset_0 [order 1] : [FLOOR==0]
          OpCl_doors.OpCl_0.Closing0.Reset.Reset_0 -> (junction 68936)
          (junction 68935) -> (junction 68937) [order 2]
          (junction 68936) -> (junction 68938)
          (junction 68937) -> OpCl_doors.OpCl_0.Closing0.Reset.Reset_1 [order 1] : [FLOOR==1]
          OpCl_doors.OpCl_0.Closing0.Reset.Reset_1 -> (junction 68938)
          (junction 68937) -> (junction 68939) [order 2]
          (junction 68938) -> (junction 68940)
          (junction 68939) -> OpCl_doors.OpCl_0.Closing0.Reset.Reset_2 [order 1] : [FLOOR==2]
          OpCl_doors.OpCl_0.Closing0.Reset.Reset_2 -> (junction 68940)
          (junction 68939) -> (junction 68941) [order 2]
          (junction 68940) -> (junction 68942)
          (junction 68941) -> OpCl_doors.OpCl_0.Closing0.Reset.Reset_3 [order 1] : [FLOOR==3]
          OpCl_doors.OpCl_0.Closing0.Reset.Reset_3 -> (junction 68942)
          (junction 68941) -> (junction 68943) [order 2]
          (junction 68942) -> (junction 68944)
          (junction 68944) -> (junction 68943)
        state Timer_close
          state Set_tmr
            en: Q_cl=true;
          state Set
            en:PT_cl=5;
            IN_cl=true;
          state Counting
            en:ET_cl = ET_cl + 1;
            Q_cl=false;
          (junction 68968) -> OpCl_doors.OpCl_0.Closing0.Timer_close.Set_tmr [order 1] : [ET_cl==PT_cl]
          OpCl_doors.OpCl_0.Closing0.Timer_close.Set_tmr -> (junction 68969)
          (default) -> OpCl_doors.OpCl_0.Closing0.Timer_close.Set
          OpCl_doors.OpCl_0.Closing0.Timer_close.Counting -> (junction 68968)
          (junction 68968) -> (junction 68969) [order 2]
          OpCl_doors.OpCl_0.Closing0.Timer_close.Set -> (junction 68970)
          (junction 68970) -> OpCl_doors.OpCl_0.Closing0.Timer_close.Counting [order 1] : [ET_cl<PT_cl]
          (junction 68970) -> (junction 68969) [order 2]
        state Closing
          en: CP0=Q_cl;
        state Button_detection
          state Save_energy
            en:
            LL=not(Q_LL);
          state Timer_LL
            state Set_tmr
              en:
              Q_LL=true;
            state Counting
              en:
              ET_LL= ET_LL + 1;
              Q_LL=false;
            state Set
              en:
              IN_LL=true;
              PT_LL=10;
            (junction 69052) -> OpCl_doors.OpCl_0.Closing0.Button_detection.Timer_LL.Set_tmr [order 1] : [ET_LL==PT_LL]
            OpCl_doors.OpCl_0.Closing0.Button_detection.Timer_LL.Set_tmr -> (junction 69053)
            OpCl_doors.OpCl_0.Closing0.Button_detection.Timer_LL.Counting -> (junction 69052)
            (junction 69052) -> (junction 69053) [order 2]
            (default) -> OpCl_doors.OpCl_0.Closing0.Button_detection.Timer_LL.Set
            OpCl_doors.OpCl_0.Closing0.Button_detection.Timer_LL.Set -> (junction 69054)
            (junction 69054) -> OpCl_doors.OpCl_0.Closing0.Button_detection.Timer_LL.Counting [order 1] : [ET_LL<PT_LL]
            (junction 69054) -> (junction 69053) [order 2]
          state BUTTON_DOWN
            state Button_DOWN_1
              en:
              BUTTON_DOWN(2)=true;
              BUT_TEMP=1;
              LPD1=true;
              PUSHED=true;
              UPDATE=false;
              IN_LL=false; ET_LL=0;
            state First_but_1
              en:
              BUT_1=BUT_TEMP;
              FIRST_BUT=false;
            state Button_DOWN_2
              en:
              BUTTON_DOWN(3)=true;
              BUT_TEMP=2;
              LPD2=true;
              PUSHED=true;
              UPDATE=false;
              IN_LL=false; ET_LL=0;
            state First_but_2
              en:
              BUT_1=BUT_TEMP;
              FIRST_BUT=false;
            state Button_DOWN_3
              en:
              BUTTON_DOWN(4)=true;
              BUT_TEMP=3;
              LPD3=true;
              PUSHED=true;
              UPDATE=false;
              IN_LL=false; ET_LL=0;
            state First_but_3
              en:
              BUT_1=BUT_TEMP;
              FIRST_BUT=false;
            (default) -> (junction 69067)
            (junction 69067) -> OpCl_doors.OpCl_0.Closing0.Button_detection.BUTTON_DOWN.Button_DOWN_1 [order 1] : [PD1]
            OpCl_doors.OpCl_0.Closing0.Button_detection.BUTTON_DOWN.Button_DOWN_1 -> (junction 69068)
            (junction 69068) -> OpCl_doors.OpCl_0.Closing0.Button_detection.BUTTON_DOWN.First_but_1 [order 1] : [FIRST_BUT && not(RPC1)]
            OpCl_doors.OpCl_0.Closing0.Button_detection.BUTTON_DOWN.First_but_1 -> (junction 69069)
            (junction 69067) -> (junction 69070) [order 2]
            (junction 69068) -> (junction 69071) [order 2]
            (junction 69069) -> (junction 69072)
            (junction 69071) -> (junction 69070)
            (junction 69072) -> (junction 69071)
            (junction 69070) -> (junction 69073)
            (junction 69073) -> OpCl_doors.OpCl_0.Closing0.Button_detection.BUTTON_DOWN.Button_DOWN_2 [order 1] : [PD2]
            OpCl_doors.OpCl_0.Closing0.Button_detection.BUTTON_DOWN.Button_DOWN_2 -> (junction 69074)
            (junction 69074) -> OpCl_doors.OpCl_0.Closing0.Button_detection.BUTTON_DOWN.First_but_2 [order 1] : [FIRST_BUT && not(RPC2)]
            OpCl_doors.OpCl_0.Closing0.Button_detection.BUTTON_DOWN.First_but_2 -> (junction 69075)
            (junction 69073) -> (junction 69076) [order 2]
            (junction 69074) -> (junction 69077) [order 2]
            (junction 69075) -> (junction 69078)
            (junction 69077) -> (junction 69076)
            (junction 69078) -> (junction 69077)
            (junction 69076) -> (junction 69079)
            (junction 69079) -> OpCl_doors.OpCl_0.Closing0.Button_detection.BUTTON_DOWN.Button_DOWN_3 [order 1] : [PD3]
            OpCl_doors.OpCl_0.Closing0.Button_detection.BUTTON_DOWN.Button_DOWN_3 -> (junction 69080)
            (junction 69080) -> OpCl_doors.OpCl_0.Closing0.Button_detection.BUTTON_DOWN.First_but_3 [order 1] : [FIRST_BUT && not(RPC3)]
            OpCl_doors.OpCl_0.Closing0.Button_detection.BUTTON_DOWN.First_but_3 -> (junction 69081)
            (junction 69079) -> (junction 69082) [order 2]
            (junction 69080) -> (junction 69083) [order 2]
            (junction 69081) -> (junction 69084)
            (junction 69083) -> (junction 69082)
            (junction 69084) -> (junction 69083)
          state BUTTON_CAR
            state Button_CAR_0
              en:
              BUTTON_CAR(1)=true;
              BUT_TEMP=0;
              LPC0=true;
              PUSHED=true;
              UPDATE=false;
              IN_LL=false; ET_LL=0;
            state First_but_0
              en:
              BUT_1=BUT_TEMP;
              FIRST_BUT=false;
            state Button_CAR_1
              en:
              BUTTON_CAR(2)=true;
              BUT_TEMP=1;
              LPC1=true;
              PUSHED=true;
              UPDATE=false;
              IN_LL=false; ET_LL=0;
            state First_but_1
              en:
              BUT_1=BUT_TEMP;
              FIRST_BUT=false;
            state Button_CAR_2
              en:
              BUTTON_CAR(3)=true;
              BUT_TEMP=2;
              LPC2=true;
              PUSHED=true;
              UPDATE=false;
              IN_LL=false; ET_LL=0;
            state First_but_2
              en:
              BUT_1=BUT_TEMP;
              FIRST_BUT=false;
            state Button_CAR_3
              en:
              BUTTON_CAR(4)=true;
              BUT_TEMP=3;
              LPC3=true;
              PUSHED=true;
              UPDATE=false;
              IN_LL=false; ET_LL=0;
            state First_but_3
              en:
              BUT_1=BUT_TEMP;
              FIRST_BUT=false;
            (default) -> (junction 69122)
            (junction 69122) -> OpCl_doors.OpCl_0.Closing0.Button_detection.BUTTON_CAR.Button_CAR_0 [order 1] : [P0]
            OpCl_doors.OpCl_0.Closing0.Button_detection.BUTTON_CAR.Button_CAR_0 -> (junction 69123)
            (junction 69123) -> OpCl_doors.OpCl_0.Closing0.Button_detection.BUTTON_CAR.First_but_0 [order 1] : [FIRST_BUT && not(RPC0)]
            OpCl_doors.OpCl_0.Closing0.Button_detection.BUTTON_CAR.First_but_0 -> (junction 69124)
            (junction 69122) -> (junction 69125) [order 2]
            (junction 69123) -> (junction 69126) [order 2]
            (junction 69124) -> (junction 69127)
            (junction 69126) -> (junction 69125)
            (junction 69127) -> (junction 69126)
            (junction 69125) -> (junction 69130)
            OpCl_doors.OpCl_0.Closing0.Button_detection.BUTTON_CAR.Button_CAR_1 -> (junction 69128)
            (junction 69128) -> OpCl_doors.OpCl_0.Closing0.Button_detection.BUTTON_CAR.First_but_1 [order 1] : [FIRST_BUT && not(RPC1)]
            OpCl_doors.OpCl_0.Closing0.Button_detection.BUTTON_CAR.First_but_1 -> (junction 69129)
            (junction 69128) -> (junction 69132) [order 2]
            (junction 69129) -> (junction 69133)
            (junction 69130) -> OpCl_doors.OpCl_0.Closing0.Button_detection.BUTTON_CAR.Button_CAR_1 [order 1] : [P1]
            (junction 69130) -> (junction 69131) [order 2]
            (junction 69132) -> (junction 69131)
            (junction 69133) -> (junction 69132)
            (junction 69131) -> (junction 69134)
            (junction 69134) -> OpCl_doors.OpCl_0.Closing0.Button_detection.BUTTON_CAR.Button_CAR_2 [order 1] : [P2]
            OpCl_doors.OpCl_0.Closing0.Button_detection.BUTTON_CAR.Button_CAR_2 -> (junction 69135)
            (junction 69135) -> OpCl_doors.OpCl_0.Closing0.Button_detection.BUTTON_CAR.First_but_2 [order 1] : [FIRST_BUT && not(RPC2)]
            OpCl_doors.OpCl_0.Closing0.Button_detection.BUTTON_CAR.First_but_2 -> (junction 69136)
            (junction 69134) -> (junction 69137) [order 2]
            (junction 69135) -> (junction 69138) [order 2]
            (junction 69136) -> (junction 69139)
            (junction 69138) -> (junction 69137)
            (junction 69139) -> (junction 69138)
            (junction 69137) -> (junction 69140)
            (junction 69140) -> OpCl_doors.OpCl_0.Closing0.Button_detection.BUTTON_CAR.Button_CAR_3 [order 1] : [P3]
            OpCl_doors.OpCl_0.Closing0.Button_detection.BUTTON_CAR.Button_CAR_3 -> (junction 69141)
            (junction 69141) -> OpCl_doors.OpCl_0.Closing0.Button_detection.BUTTON_CAR.First_but_3 [order 1] : [FIRST_BUT && not(RPC3)]
            OpCl_doors.OpCl_0.Closing0.Button_detection.BUTTON_CAR.First_but_3 -> (junction 69142)
            (junction 69140) -> (junction 69143) [order 2]
            (junction 69141) -> (junction 69144) [order 2]
            (junction 69142) -> (junction 69145)
            (junction 69144) -> (junction 69143)
            (junction 69145) -> (junction 69144)
          state BUTTON_UP
            state Button_UP_0
              en:
              BUTTON_UP(1)=true;
              BUT_TEMP=0;
              LPS0=true;
              PUSHED=true;
              UPDATE=false;
              IN_LL=false; ET_LL=0;
            state First_but_0
              en:
              BUT_1=BUT_TEMP;
              FIRST_BUT=false;
            state Button_UP_1
              en:
              BUTTON_UP(2)=true;
              BUT_TEMP=1;
              LPS1=true;
              PUSHED=true;
              UPDATE=false;
              IN_LL=false; ET_LL=0;
            state First_but_1
              en:
              BUT_1=BUT_TEMP;
              FIRST_BUT=false;
            state Button_UP_2
              en:
              BUTTON_UP(3)=true;
              BUT_TEMP=2;
              LPS2=true;
              PUSHED=true;
              UPDATE=false;
              IN_LL=false; ET_LL=0;
            state First_but_2
              en:
              BUT_1=BUT_TEMP;
              FIRST_BUT=false;
            (junction 69195) -> OpCl_doors.OpCl_0.Closing0.Button_detection.BUTTON_UP.Button_UP_0 [order 1] : [PS0]
            OpCl_doors.OpCl_0.Closing0.Button_detection.BUTTON_UP.Button_UP_0 -> (junction 69196)
            (junction 69196) -> OpCl_doors.OpCl_0.Closing0.Button_detection.BUTTON_UP.First_but_0 [order 1] : [FIRST_BUT && not(RPC0)]
            OpCl_doors.OpCl_0.Closing0.Button_detection.BUTTON_UP.First_but_0 -> (junction 69197)
            (default) -> (junction 69195)
            (junction 69195) -> (junction 69200) [order 2]
            (junction 69196) -> (junction 69198) [order 2]
            (junction 69197) -> (junction 69199)
            (junction 69199) -> (junction 69198)
            (junction 69198) -> (junction 69200)
            (junction 69200) -> (junction 69201)
            (junction 69201) -> OpCl_doors.OpCl_0.Closing0.Button_detection.BUTTON_UP.Button_UP_1 [order 1] : [PS1]
            OpCl_doors.OpCl_0.Closing0.Button_detection.BUTTON_UP.Button_UP_1 -> (junction 69202)
            (junction 69202) -> OpCl_doors.OpCl_0.Closing0.Button_detection.BUTTON_UP.First_but_1 [order 1] : [FIRST_BUT && not(RPC1)]
            OpCl_doors.OpCl_0.Closing0.Button_detection.BUTTON_UP.First_but_1 -> (junction 69203)
            (junction 69201) -> (junction 69204) [order 2]
            (junction 69202) -> (junction 69205) [order 2]
            (junction 69203) -> (junction 69206)
            (junction 69205) -> (junction 69204)
            (junction 69206) -> (junction 69205)
            (junction 69204) -> (junction 69208)
            OpCl_doors.OpCl_0.Closing0.Button_detection.BUTTON_UP.First_but_2 -> (junction 69207)
            (junction 69207) -> (junction 69212)
            (junction 69208) -> OpCl_doors.OpCl_0.Closing0.Button_detection.BUTTON_UP.Button_UP_2 [order 1] : [PS2]
            OpCl_doors.OpCl_0.Closing0.Button_detection.BUTTON_UP.Button_UP_2 -> (junction 69209)
            (junction 69209) -> OpCl_doors.OpCl_0.Closing0.Button_detection.BUTTON_UP.First_but_2 [order 1] : [FIRST_BUT && not(RPC2)]
            (junction 69208) -> (junction 69210) [order 2]
            (junction 69209) -> (junction 69211) [order 2]
            (junction 69211) -> (junction 69210)
            (junction 69212) -> (junction 69211)
          state Max_Min_assignment
            state Min_but
              en:
              BUTTON=MIN_BUT;
            state Max_but
              en:
              BUTTON=MAX_BUT;
            state First_but
              en:
              BUTTON=BUT_1;
            state Max_but1
              en:
              MAX_BUT=2;
            state Max_but2
              en:
              MAX_BUT=1;
            state Max_but3
              en:
              MAX_BUT=0;
            state Min_but1
              en:
              MIN_BUT=1;
            state Min_but2
              en:
              MIN_BUT=2;
            state Min_but3
              en:
              MIN_BUT=3;
            state MAX
              en:
              MAX_BUT=BUT_TEMP;
            state MIN
              en:
              MIN_BUT=BUT_TEMP;
            state Updating_button_0
              en:
              BUTTON=MAX_BUT;
            state Updating_button_1
              en:
              BUTTON=MIN_BUT;
            (junction 69250) -> OpCl_doors.OpCl_0.Closing0.Button_detection.Max_Min_assignment.Min_but [order 1] : [(MAX_BUT-FLOOR)>(FLOOR-MIN_BUT)]
            OpCl_doors.OpCl_0.Closing0.Button_detection.Max_Min_assignment.Min_but -> (junction 69251)
            (junction 69252) -> (junction 69250) [order 1] : [not(FLAG_STOP) && MOTION==2 && FLAG==3]
            (default) -> (junction 69252)
            (junction 69250) -> (junction 69253) [order 2]
            (junction 69251) -> (junction 69254)
            (junction 69252) -> (junction 69255) [order 2]
            (junction 69253) -> OpCl_doors.OpCl_0.Closing0.Button_detection.Max_Min_assignment.Max_but [order 1] : [(MAX_BUT-FLOOR)<(FLOOR-MIN_BUT)]
            OpCl_doors.OpCl_0.Closing0.Button_detection.Max_Min_assignment.Max_but -> (junction 69254)
            (junction 69253) -> OpCl_doors.OpCl_0.Closing0.Button_detection.Max_Min_assignment.First_but [order 2]
            (junction 69254) -> (junction 69257)
            OpCl_doors.OpCl_0.Closing0.Button_detection.Max_Min_assignment.First_but -> (junction 69256)
            (junction 69256) -> (junction 69255)
            (junction 69257) -> (junction 69256)
            (junction 69255) -> (junction 69258)
            (junction 69259) -> (junction 69260) [order 1] : [MOTION==0]
                | {MOTION=1;
                | UPDATE=true;}
            (junction 69260) -> OpCl_doors.OpCl_0.Closing0.Button_detection.Max_Min_assignment.Max_but1 [order 1] : [BUTTON_UP(2)]
            OpCl_doors.OpCl_0.Closing0.Button_detection.Max_Min_assignment.Max_but1 -> (junction 69261)
            (junction 69258) -> (junction 69259) [order 1] : [BUTTON==FLOOR && EXTEND]
                | {EXTEND=false;}
            (junction 69258) -> (junction 69272) [order 2]
            (junction 69259) -> (junction 69264) [order 2]
            (junction 69260) -> (junction 69262) [order 2]
            (junction 69261) -> (junction 69263)
            (junction 69262) -> OpCl_doors.OpCl_0.Closing0.Button_detection.Max_Min_assignment.Max_but2 [order 1] : [BUTTON_UP(1)]
            OpCl_doors.OpCl_0.Closing0.Button_detection.Max_Min_assignment.Max_but2 -> (junction 69263)
            (junction 69262) -> OpCl_doors.OpCl_0.Closing0.Button_detection.Max_Min_assignment.Max_but3 [order 2]
            (junction 69263) -> (junction 69266)
            OpCl_doors.OpCl_0.Closing0.Button_detection.Max_Min_assignment.Max_but3 -> (junction 69265)
            (junction 69265) -> (junction 69264)
            (junction 69266) -> (junction 69265)
            (junction 69264) -> (junction 69267)
            (junction 69267) -> (junction 69268) [order 1] : [MOTION==1]
                | {MOTION=0;
                | UPDATE=true;}
            (junction 69268) -> OpCl_doors.OpCl_0.Closing0.Button_detection.Max_Min_assignment.Min_but1 [order 1] : [BUTTON_DOWN(1)]
            OpCl_doors.OpCl_0.Closing0.Button_detection.Max_Min_assignment.Min_but1 -> (junction 69269)
            (junction 69267) -> (junction 69273) [order 2]
            (junction 69268) -> (junction 69270) [order 2]
            (junction 69269) -> (junction 69271)
            (junction 69270) -> OpCl_doors.OpCl_0.Closing0.Button_detection.Max_Min_assignment.Min_but2 [order 1] : [BUTTON_DOWN(2)]
            OpCl_doors.OpCl_0.Closing0.Button_detection.Max_Min_assignment.Min_but2 -> (junction 69271)
            (junction 69270) -> OpCl_doors.OpCl_0.Closing0.Button_detection.Max_Min_assignment.Min_but3 [order 2]
            (junction 69271) -> (junction 69275)
            OpCl_doors.OpCl_0.Closing0.Button_detection.Max_Min_assignment.Min_but3 -> (junction 69274)
            (junction 69273) -> (junction 69272)
            (junction 69274) -> (junction 69273)
            (junction 69275) -> (junction 69274)
            (junction 69272) -> (junction 69277)
            OpCl_doors.OpCl_0.Closing0.Button_detection.Max_Min_assignment.MAX -> (junction 69276)
            (junction 69277) -> (junction 69278) [order 1] : [PUSHED]
            (junction 69278) -> (junction 69279) [order 1] : [not(BUT_TEMP==FLOOR) || not(MOTION==2)]
            (junction 69279) -> OpCl_doors.OpCl_0.Closing0.Button_detection.Max_Min_assignment.MAX [order 1] : [MAX_BUT<BUT_TEMP && not(UPDATE)]
            (junction 69276) -> (junction 69281)
            (junction 69277) -> (junction 69291) [order 2]
            (junction 69278) -> (junction 69284) [order 2]
            (junction 69279) -> (junction 69280) [order 2]
            (junction 69281) -> (junction 69280)
            (junction 69280) -> (junction 69282)
            (junction 69282) -> OpCl_doors.OpCl_0.Closing0.Button_detection.Max_Min_assignment.MIN [order 1] : [MIN_BUT>BUT_TEMP && not(UPDATE)]
            OpCl_doors.OpCl_0.Closing0.Button_detection.Max_Min_assignment.MIN -> (junction 69283)
            (junction 69282) -> (junction 69285) [order 2]
            (junction 69283) -> (junction 69286)
            (junction 69285) -> (junction 69284)
            (junction 69286) -> (junction 69285)
            (junction 69284) -> (junction 69287)
            (junction 69287) -> OpCl_doors.OpCl_0.Closing0.Button_detection.Max_Min_assignment.Updating_button_0 [order 1] : [MOTION==0]
            OpCl_doors.OpCl_0.Closing0.Button_detection.Max_Min_assignment.Updating_button_0 -> (junction 69288)
            (junction 69287) -> (junction 69289) [order 2]
            (junction 69288) -> (junction 69290)
            (junction 69289) -> OpCl_doors.OpCl_0.Closing0.Button_detection.Max_Min_assignment.Updating_button_1 [order 1] : [MOTION==1]
            OpCl_doors.OpCl_0.Closing0.Button_detection.Max_Min_assignment.Updating_button_1 -> (junction 69290)
            (junction 69289) -> (junction 69292) [order 2]
            (junction 69290) -> (junction 69293)
            (junction 69292) -> (junction 69291)
            (junction 69293) -> (junction 69292)
          state GoTo_PositionControl
            en:
            BUTTON=BUT_TEMP;
            FLAG=2;
          state Emergency
            en:
            FLAG_EMG=true;
            FLAG=4;
          state Timer_EME
            state Set_tmr
              en:
              Q_EME=true;
            state Counting
              en:
              ET_EME= ET_EME + 1;
              Q_EME=false;
            state Set
              en:
              IN_EME=true;
              PT_EME=3;
            (junction 69383) -> OpCl_doors.OpCl_0.Closing0.Button_detection.Timer_EME.Set_tmr [order 1] : [ET_EME==PT_EME]
            OpCl_doors.OpCl_0.Closing0.Button_detection.Timer_EME.Set_tmr -> (junction 69384)
            OpCl_doors.OpCl_0.Closing0.Button_detection.Timer_EME.Counting -> (junction 69383)
            (junction 69383) -> (junction 69384) [order 2]
            (default) -> OpCl_doors.OpCl_0.Closing0.Button_detection.Timer_EME.Set
            OpCl_doors.OpCl_0.Closing0.Button_detection.Timer_EME.Set -> (junction 69385)
            (junction 69385) -> OpCl_doors.OpCl_0.Closing0.Button_detection.Timer_EME.Counting [order 1] : [ET_EME<PT_EME]
            (junction 69385) -> (junction 69384) [order 2]
          state Not_Emergency
            en:
            IN_EME=false;
            ET_EME=0;
          state SwitchingOFF_LEDs
            en:
            LPD3=false;
            LPD2=false;
            LPS2=false;
            LPD1=false;
            LPS1=false;
            LPS0=false;
          (default) -> (junction 68984)
          (junction 68984) -> (junction 68985) [order 1] : [FLAG==1 && not(PUSHED)]
              | {BUTTON=FLOOR;
              | BUT_TEMP=BUTTON;
              | BUT_1=FLOOR;}
          (junction 68985) -> OpCl_doors.OpCl_0.Closing0.Button_detection.Timer_LL [order 1] : [not(FLAG_STOP)]
          OpCl_doors.OpCl_0.Closing0.Button_detection.Save_energy -> (junction 68986)
          OpCl_doors.OpCl_0.Closing0.Button_detection.Timer_LL -> OpCl_doors.OpCl_0.Closing0.Button_detection.Save_energy
          (junction 68985) -> (junction 68988) [order 2]
          (junction 68984) -> (junction 68987) [order 2]
          (junction 68986) -> (junction 68989)
          (junction 68988) -> (junction 68987)
          (junction 68989) -> (junction 68988)
          (junction 68987) -> OpCl_doors.OpCl_0.Closing0.Button_detection.BUTTON_CAR
          OpCl_doors.OpCl_0.Closing0.Button_detection.BUTTON_UP -> OpCl_doors.OpCl_0.Closing0.Button_detection.BUTTON_DOWN
          OpCl_doors.OpCl_0.Closing0.Button_detection.BUTTON_DOWN -> OpCl_doors.OpCl_0.Closing0.Button_detection.Max_Min_assignment
          OpCl_doors.OpCl_0.Closing0.Button_detection.Max_Min_assignment -> (junction 68990)
          OpCl_doors.OpCl_0.Closing0.Button_detection.BUTTON_CAR -> OpCl_doors.OpCl_0.Closing0.Button_detection.BUTTON_UP
          (junction 68990) -> (junction 68992)
          (junction 68992) -> (junction 68991)
          (junction 68991) -> (junction 68994)
          OpCl_doors.OpCl_0.Closing0.Button_detection.GoTo_PositionControl -> (junction 68993)
          (junction 68994) -> (junction 68995) [order 1] : [FLAG==1]
          (junction 68995) -> OpCl_doors.OpCl_0.Closing0.Button_detection.GoTo_PositionControl [order 1] : [PUSHED]
          (junction 68993) -> (junction 68997)
          (junction 68994) -> (junction 69005) [order 2]
          (junction 68995) -> (junction 68996) [order 2]
          (junction 68997) -> (junction 68996)
          (junction 68996) -> (junction 68999)
          OpCl_doors.OpCl_0.Closing0.Button_detection.Emergency -> (junction 68998)
          (junction 68999) -> OpCl_doors.OpCl_0.Closing0.Button_detection.Timer_EME [order 1] : [STOP]
              | {IN_LL=false; ET_LL=0;FLAG=1;}
          OpCl_doors.OpCl_0.Closing0.Button_detection.Timer_EME -> (junction 69000)
          (junction 69000) -> OpCl_doors.OpCl_0.Closing0.Button_detection.Emergency [order 1] : [Q_EME]
          (junction 68998) -> (junction 69002)
          (junction 68999) -> OpCl_doors.OpCl_0.Closing0.Button_detection.Not_Emergency [order 2]
          (junction 69000) -> (junction 69001) [order 2]
          (junction 69002) -> (junction 69001)
          (junction 69001) -> (junction 69004)
          OpCl_doors.OpCl_0.Closing0.Button_detection.Not_Emergency -> (junction 69004)
          OpCl_doors.OpCl_0.Closing0.Button_detection.SwitchingOFF_LEDs -> (junction 69003)
          (junction 69004) -> OpCl_doors.OpCl_0.Closing0.Button_detection.SwitchingOFF_LEDs [order 1] : [FLAG_STOP && FLAG==2]
          (junction 69003) -> (junction 69007)
          (junction 69004) -> (junction 69006) [order 2]
          (junction 69006) -> (junction 69005)
          (junction 69007) -> (junction 69006)
        state Extending
          en:
          EXTEND=true;
        state Stop_Closing
          en:
          CP0=false;
          FLAG_OD=false;
          OBS=false;
          ET_cl=0;
          IN_cl=false;
        state GoTo_PositionControl
          en: FLAG=2;
        state GoTo_BUttonDetection
          en:
          MOTION=2;
          MAX_BUT=0;
          MIN_BUT=3;
          PUSHED=false;
          FIRST_BUT=true;
          FLAG=1;
          UPDATE=false;
        state Closing1
          en:CP0=true;
        state Stop_Closing1
          en:CP0=false;
        OpCl_doors.OpCl_0.Closing0.Reset -> OpCl_doors.OpCl_0.Closing0.Timer_close
        (default) -> (junction 68895)
        (junction 68895) -> OpCl_doors.OpCl_0.Closing0.Reset [order 1] : [not(FLAG==0) && not(FLAG==4)]
        OpCl_doors.OpCl_0.Closing0.Timer_close -> (junction 68896)
        (junction 68896) -> OpCl_doors.OpCl_0.Closing0.Closing [order 1] : [not(PC0)]
        OpCl_doors.OpCl_0.Closing0.Button_detection -> (junction 68897)
        OpCl_doors.OpCl_0.Closing0.Closing -> OpCl_doors.OpCl_0.Closing0.Button_detection
        (junction 68895) -> (junction 68905) [order 2]
        (junction 68896) -> (junction 68898) [order 2]
        (junction 68897) -> (junction 68903)
        (junction 68898) -> OpCl_doors.OpCl_0.Closing0.Extending [order 1] : [BUTTON==FLOOR]
        (junction 68898) -> (junction 68900) [order 2]
        OpCl_doors.OpCl_0.Closing0.Extending -> (junction 68899)
        (junction 68899) -> (junction 68900)
        (junction 68900) -> OpCl_doors.OpCl_0.Closing0.Stop_Closing
        OpCl_doors.OpCl_0.Closing0.Stop_Closing -> (junction 68901)
        (junction 68901) -> OpCl_doors.OpCl_0.Closing0.GoTo_PositionControl [order 2]
        (junction 68901) -> OpCl_doors.OpCl_0.Closing0.GoTo_BUttonDetection [order 1] : [not(BUTTON_CAR(1) || BUTTON_CAR(2) || BUTTON_CAR(3) || BUTTON_CAR(4) || BUTTON_UP(1) || BUTTON_UP(2) || BUTTON_UP(3) || BUTTON_DOWN(2) || BUTTON_DOWN(3) || BUTTON_DOWN(4))]
        OpCl_doors.OpCl_0.Closing0.GoTo_PositionControl -> (junction 68902)
        OpCl_doors.OpCl_0.Closing0.GoTo_BUttonDetection -> (junction 68902)
        (junction 68902) -> (junction 68903)
        (junction 68903) -> (junction 68904)
        (junction 68904) -> (junction 68906)
        (junction 68905) -> OpCl_doors.OpCl_0.Closing0.Closing1 [order 1] : [not(PC0)]
        OpCl_doors.OpCl_0.Closing0.Closing1 -> (junction 68906)
        (junction 68905) -> OpCl_doors.OpCl_0.Closing0.Stop_Closing1 [order 2]
        OpCl_doors.OpCl_0.Closing0.Stop_Closing1 -> (junction 68906)
      state StopClosing
        en: CP0=false;
        FLAG_OD=false;
      state Opening0
        state Opening
          en:AP0=Q_op;
        state People_IN
          state Check_People_IN
            en:
            COUNTER_IN=false;
          state People_KID_IN
            en:
            WEIGHT=WEIGHT+30;
            KIDS=KIDS+1;
          state People_WOMAN_IN
            en:
            WEIGHT=WEIGHT+55;
            WOMEN=WOMEN+1;
          state People_MAN_IN
            en:
            WEIGHT=WEIGHT+75;
            MEN=MEN+1;
          state People_FATGUY_IN
            en:
            WEIGHT=WEIGHT+100;
            FATGUYS=FATGUYS+1;
          state Re_Ready_IN
            en:
            COUNTER_IN=true;
          (default) -> (junction 30509)
          (junction 30509) -> OpCl_doors.OpCl_0.Opening0.People_IN.Check_People_IN [order 1] : [COUNTER_IN]
          OpCl_doors.OpCl_0.Opening0.People_IN.Check_People_IN -> (junction 12612)
          (junction 12612) -> OpCl_doors.OpCl_0.Opening0.People_IN.People_KID_IN [order 1] : [KID_IN]
          OpCl_doors.OpCl_0.Opening0.People_IN.People_KID_IN -> (junction 30513)
          (junction 30509) -> (junction 30533) [order 2]
          (junction 12612) -> (junction 30511) [order 2]
          (junction 30513) -> (junction 30514)
          (junction 30511) -> OpCl_doors.OpCl_0.Opening0.People_IN.People_WOMAN_IN [order 1] : [WOMAN_IN]
          OpCl_doors.OpCl_0.Opening0.People_IN.People_WOMAN_IN -> (junction 30514)
          (junction 30511) -> (junction 30518) [order 2]
          (junction 30514) -> (junction 30520)
          (junction 30518) -> OpCl_doors.OpCl_0.Opening0.People_IN.People_MAN_IN [order 1] : [MAN_IN]
          OpCl_doors.OpCl_0.Opening0.People_IN.People_MAN_IN -> (junction 30520)
          (junction 30518) -> (junction 30523) [order 2]
          (junction 30520) -> (junction 30525)
          (junction 30523) -> OpCl_doors.OpCl_0.Opening0.People_IN.People_FATGUY_IN [order 1] : [FATGUY_IN]
          OpCl_doors.OpCl_0.Opening0.People_IN.People_FATGUY_IN -> (junction 30525)
          (junction 30523) -> (junction 30528) [order 2]
          (junction 30525) -> (junction 30531)
          (junction 30528) -> (junction 30533)
          (junction 30531) -> (junction 30528)
          (junction 30533) -> (junction 30540)
          (junction 30540) -> OpCl_doors.OpCl_0.Opening0.People_IN.Re_Ready_IN [order 1] : [not(KID_IN|| WOMAN_IN || MAN_IN || FATGUY_IN)]
          (junction 30540) -> (junction 30542) [order 2]
          OpCl_doors.OpCl_0.Opening0.People_IN.Re_Ready_IN -> (junction 30544)
          (junction 30544) -> (junction 30542)
        state Timer_open
          state Set_tmr
            en: Q_op=true;
          state Set
            en:PT_op=2;
            IN_op=true;
          state Counting
            en:ET_op = ET_op + 1;
            Q_op=false;
          (junction 12585) -> OpCl_doors.OpCl_0.Opening0.Timer_open.Set_tmr [order 1] : [ET_op==PT_op]
          OpCl_doors.OpCl_0.Opening0.Timer_open.Set_tmr -> (junction 12586)
          (default) -> OpCl_doors.OpCl_0.Opening0.Timer_open.Set
          OpCl_doors.OpCl_0.Opening0.Timer_open.Counting -> (junction 12585)
          (junction 12585) -> (junction 12586) [order 2]
          OpCl_doors.OpCl_0.Opening0.Timer_open.Set -> (junction 12587)
          (junction 12587) -> OpCl_doors.OpCl_0.Opening0.Timer_open.Counting [order 1] : [ET_op<PT_op]
          (junction 12587) -> (junction 12586) [order 2]
        state Stop_Opening
          en:AP0=false;
          FLAG_OD=true;
          OBS=true;
          IN_op=false;
          ET_op=0;
        state People_OUT
          state Check_People_OUT
            en:
            COUNTER_OUT=false;
          state People_KID_OUT
            en:
            WEIGHT=WEIGHT-30;
            KIDS=KIDS-1;
          state People_WOMAN_OUT
            en:
            WEIGHT=WEIGHT-55;
            WOMEN=WOMEN-1;
          state People_MAN_OUT
            en:
            WEIGHT=WEIGHT-75;
            MEN=MEN-1;
          state People_FATGUY_OUT
            en:
            WEIGHT=WEIGHT-100;
            FATGUYS=FATGUYS-1;
          state Re_Ready_OUT
            en:
            COUNTER_OUT=true;
          (default) -> (junction 30549)
          (junction 30549) -> OpCl_doors.OpCl_0.Opening0.People_OUT.Check_People_OUT [order 1] : [COUNTER_OUT]
          OpCl_doors.OpCl_0.Opening0.People_OUT.Check_People_OUT -> (junction 12645)
          (junction 12645) -> OpCl_doors.OpCl_0.Opening0.People_OUT.People_KID_OUT [order 1] : [KID_OUT && KIDS>0 ]
          OpCl_doors.OpCl_0.Opening0.People_OUT.People_KID_OUT -> (junction 30551)
          (junction 30549) -> (junction 30575) [order 2]
          (junction 12645) -> (junction 30552) [order 2]
          (junction 30551) -> (junction 30554)
          (junction 30552) -> OpCl_doors.OpCl_0.Opening0.People_OUT.People_WOMAN_OUT [order 1] : [WOMAN_OUT && WOMEN>0]
          OpCl_doors.OpCl_0.Opening0.People_OUT.People_WOMAN_OUT -> (junction 30554)
          (junction 30554) -> (junction 30561)
          (junction 30552) -> (junction 30558) [order 2]
          (junction 30558) -> OpCl_doors.OpCl_0.Opening0.People_OUT.People_MAN_OUT [order 1] : [MAN_OUT && MEN>0]
          OpCl_doors.OpCl_0.Opening0.People_OUT.People_MAN_OUT -> (junction 30561)
          (junction 30558) -> (junction 30564) [order 2]
          (junction 30561) -> (junction 30566)
          (junction 30564) -> OpCl_doors.OpCl_0.Opening0.People_OUT.People_FATGUY_OUT [order 1] : [FATGUY_OUT && FATGUYS>0]
          OpCl_doors.OpCl_0.Opening0.People_OUT.People_FATGUY_OUT -> (junction 30566)
          (junction 30564) -> (junction 30568) [order 2]
          (junction 30566) -> (junction 30569)
          (junction 30568) -> (junction 30575)
          (junction 30569) -> (junction 30568)
          (junction 30575) -> (junction 30582)
          (junction 30582) -> OpCl_doors.OpCl_0.Opening0.People_OUT.Re_Ready_OUT [order 1] : [not(KID_OUT || WOMAN_OUT || MAN_OUT || FATGUY_OUT)]
          (junction 30582) -> (junction 30585) [order 2]
          OpCl_doors.OpCl_0.Opening0.People_OUT.Re_Ready_OUT -> (junction 30587)
          (junction 30587) -> (junction 30585)
        state Button_detection
          state Save_energy
            en:
            LL=not(Q_LL);
          state Timer_LL
            state Set_tmr
              en:
              Q_LL=true;
            state Counting
              en:
              ET_LL= ET_LL + 1;
              Q_LL=false;
            state Set
              en:
              IN_LL=true;
              PT_LL=10;
            (junction 71007) -> OpCl_doors.OpCl_0.Opening0.Button_detection.Timer_LL.Set_tmr [order 1] : [ET_LL==PT_LL]
            OpCl_doors.OpCl_0.Opening0.Button_detection.Timer_LL.Set_tmr -> (junction 71008)
            OpCl_doors.OpCl_0.Opening0.Button_detection.Timer_LL.Counting -> (junction 71007)
            (junction 71007) -> (junction 71008) [order 2]
            (default) -> OpCl_doors.OpCl_0.Opening0.Button_detection.Timer_LL.Set
            OpCl_doors.OpCl_0.Opening0.Button_detection.Timer_LL.Set -> (junction 71009)
            (junction 71009) -> OpCl_doors.OpCl_0.Opening0.Button_detection.Timer_LL.Counting [order 1] : [ET_LL<PT_LL]
            (junction 71009) -> (junction 71008) [order 2]
          state BUTTON_DOWN
            state Button_DOWN_1
              en:
              BUTTON_DOWN(2)=true;
              BUT_TEMP=1;
              LPD1=true;
              PUSHED=true;
              UPDATE=false;
              IN_LL=false; ET_LL=0;
            state First_but_1
              en:
              BUT_1=BUT_TEMP;
              FIRST_BUT=false;
            state Button_DOWN_2
              en:
              BUTTON_DOWN(3)=true;
              BUT_TEMP=2;
              LPD2=true;
              PUSHED=true;
              UPDATE=false;
              IN_LL=false; ET_LL=0;
            state First_but_2
              en:
              BUT_1=BUT_TEMP;
              FIRST_BUT=false;
            state Button_DOWN_3
              en:
              BUTTON_DOWN(4)=true;
              BUT_TEMP=3;
              LPD3=true;
              PUSHED=true;
              UPDATE=false;
              IN_LL=false; ET_LL=0;
            state First_but_3
              en:
              BUT_1=BUT_TEMP;
              FIRST_BUT=false;
            (default) -> (junction 71022)
            (junction 71022) -> OpCl_doors.OpCl_0.Opening0.Button_detection.BUTTON_DOWN.Button_DOWN_1 [order 1] : [PD1]
            OpCl_doors.OpCl_0.Opening0.Button_detection.BUTTON_DOWN.Button_DOWN_1 -> (junction 71023)
            (junction 71023) -> OpCl_doors.OpCl_0.Opening0.Button_detection.BUTTON_DOWN.First_but_1 [order 1] : [FIRST_BUT && not(RPC1)]
            OpCl_doors.OpCl_0.Opening0.Button_detection.BUTTON_DOWN.First_but_1 -> (junction 71024)
            (junction 71022) -> (junction 71025) [order 2]
            (junction 71023) -> (junction 71026) [order 2]
            (junction 71024) -> (junction 71027)
            (junction 71026) -> (junction 71025)
            (junction 71027) -> (junction 71026)
            (junction 71025) -> (junction 71028)
            (junction 71028) -> OpCl_doors.OpCl_0.Opening0.Button_detection.BUTTON_DOWN.Button_DOWN_2 [order 1] : [PD2]
            OpCl_doors.OpCl_0.Opening0.Button_detection.BUTTON_DOWN.Button_DOWN_2 -> (junction 71029)
            (junction 71029) -> OpCl_doors.OpCl_0.Opening0.Button_detection.BUTTON_DOWN.First_but_2 [order 1] : [FIRST_BUT && not(RPC2)]
            OpCl_doors.OpCl_0.Opening0.Button_detection.BUTTON_DOWN.First_but_2 -> (junction 71030)
            (junction 71028) -> (junction 71031) [order 2]
            (junction 71029) -> (junction 71032) [order 2]
            (junction 71030) -> (junction 71033)
            (junction 71032) -> (junction 71031)
            (junction 71033) -> (junction 71032)
            (junction 71031) -> (junction 71034)
            (junction 71034) -> OpCl_doors.OpCl_0.Opening0.Button_detection.BUTTON_DOWN.Button_DOWN_3 [order 1] : [PD3]
            OpCl_doors.OpCl_0.Opening0.Button_detection.BUTTON_DOWN.Button_DOWN_3 -> (junction 71035)
            (junction 71035) -> OpCl_doors.OpCl_0.Opening0.Button_detection.BUTTON_DOWN.First_but_3 [order 1] : [FIRST_BUT && not(RPC3)]
            OpCl_doors.OpCl_0.Opening0.Button_detection.BUTTON_DOWN.First_but_3 -> (junction 71036)
            (junction 71034) -> (junction 71037) [order 2]
            (junction 71035) -> (junction 71038) [order 2]
            (junction 71036) -> (junction 71039)
            (junction 71038) -> (junction 71037)
            (junction 71039) -> (junction 71038)
          state BUTTON_CAR
            state Button_CAR_0
              en:
              BUTTON_CAR(1)=true;
              BUT_TEMP=0;
              LPC0=true;
              PUSHED=true;
              UPDATE=false;
              IN_LL=false; ET_LL=0;
            state First_but_0
              en:
              BUT_1=BUT_TEMP;
              FIRST_BUT=false;
            state Button_CAR_1
              en:
              BUTTON_CAR(2)=true;
              BUT_TEMP=1;
              LPC1=true;
              PUSHED=true;
              UPDATE=false;
              IN_LL=false; ET_LL=0;
            state First_but_1
              en:
              BUT_1=BUT_TEMP;
              FIRST_BUT=false;
            state Button_CAR_2
              en:
              BUTTON_CAR(3)=true;
              BUT_TEMP=2;
              LPC2=true;
              PUSHED=true;
              UPDATE=false;
              IN_LL=false; ET_LL=0;
            state First_but_2
              en:
              BUT_1=BUT_TEMP;
              FIRST_BUT=false;
            state Button_CAR_3
              en:
              BUTTON_CAR(4)=true;
              BUT_TEMP=3;
              LPC3=true;
              PUSHED=true;
              UPDATE=false;
              IN_LL=false; ET_LL=0;
            state First_but_3
              en:
              BUT_1=BUT_TEMP;
              FIRST_BUT=false;
            (default) -> (junction 71077)
            (junction 71077) -> OpCl_doors.OpCl_0.Opening0.Button_detection.BUTTON_CAR.Button_CAR_0 [order 1] : [P0]
            OpCl_doors.OpCl_0.Opening0.Button_detection.BUTTON_CAR.Button_CAR_0 -> (junction 71078)
            (junction 71078) -> OpCl_doors.OpCl_0.Opening0.Button_detection.BUTTON_CAR.First_but_0 [order 1] : [FIRST_BUT && not(RPC0)]
            OpCl_doors.OpCl_0.Opening0.Button_detection.BUTTON_CAR.First_but_0 -> (junction 71079)
            (junction 71077) -> (junction 71080) [order 2]
            (junction 71078) -> (junction 71081) [order 2]
            (junction 71079) -> (junction 71082)
            (junction 71081) -> (junction 71080)
            (junction 71082) -> (junction 71081)
            (junction 71080) -> (junction 71085)
            OpCl_doors.OpCl_0.Opening0.Button_detection.BUTTON_CAR.Button_CAR_1 -> (junction 71083)
            (junction 71083) -> OpCl_doors.OpCl_0.Opening0.Button_detection.BUTTON_CAR.First_but_1 [order 1] : [FIRST_BUT && not(RPC1)]
            OpCl_doors.OpCl_0.Opening0.Button_detection.BUTTON_CAR.First_but_1 -> (junction 71084)
            (junction 71083) -> (junction 71087) [order 2]
            (junction 71084) -> (junction 71088)
            (junction 71085) -> OpCl_doors.OpCl_0.Opening0.Button_detection.BUTTON_CAR.Button_CAR_1 [order 1] : [P1]
            (junction 71085) -> (junction 71086) [order 2]
            (junction 71087) -> (junction 71086)
            (junction 71088) -> (junction 71087)
            (junction 71086) -> (junction 71089)
            (junction 71089) -> OpCl_doors.OpCl_0.Opening0.Button_detection.BUTTON_CAR.Button_CAR_2 [order 1] : [P2]
            OpCl_doors.OpCl_0.Opening0.Button_detection.BUTTON_CAR.Button_CAR_2 -> (junction 71090)
            (junction 71090) -> OpCl_doors.OpCl_0.Opening0.Button_detection.BUTTON_CAR.First_but_2 [order 1] : [FIRST_BUT && not(RPC2)]
            OpCl_doors.OpCl_0.Opening0.Button_detection.BUTTON_CAR.First_but_2 -> (junction 71091)
            (junction 71089) -> (junction 71092) [order 2]
            (junction 71090) -> (junction 71093) [order 2]
            (junction 71091) -> (junction 71094)
            (junction 71093) -> (junction 71092)
            (junction 71094) -> (junction 71093)
            (junction 71092) -> (junction 71095)
            (junction 71095) -> OpCl_doors.OpCl_0.Opening0.Button_detection.BUTTON_CAR.Button_CAR_3 [order 1] : [P3]
            OpCl_doors.OpCl_0.Opening0.Button_detection.BUTTON_CAR.Button_CAR_3 -> (junction 71096)
            (junction 71096) -> OpCl_doors.OpCl_0.Opening0.Button_detection.BUTTON_CAR.First_but_3 [order 1] : [FIRST_BUT && not(RPC3)]
            OpCl_doors.OpCl_0.Opening0.Button_detection.BUTTON_CAR.First_but_3 -> (junction 71097)
            (junction 71095) -> (junction 71098) [order 2]
            (junction 71096) -> (junction 71099) [order 2]
            (junction 71097) -> (junction 71100)
            (junction 71099) -> (junction 71098)
            (junction 71100) -> (junction 71099)
          state BUTTON_UP
            state Button_UP_0
              en:
              BUTTON_UP(1)=true;
              BUT_TEMP=0;
              LPS0=true;
              PUSHED=true;
              UPDATE=false;
              IN_LL=false; ET_LL=0;
            state First_but_0
              en:
              BUT_1=BUT_TEMP;
              FIRST_BUT=false;
            state Button_UP_1
              en:
              BUTTON_UP(2)=true;
              BUT_TEMP=1;
              LPS1=true;
              PUSHED=true;
              UPDATE=false;
              IN_LL=false; ET_LL=0;
            state First_but_1
              en:
              BUT_1=BUT_TEMP;
              FIRST_BUT=false;
            state Button_UP_2
              en:
              BUTTON_UP(3)=true;
              BUT_TEMP=2;
              LPS2=true;
              PUSHED=true;
              UPDATE=false;
              IN_LL=false; ET_LL=0;
            state First_but_2
              en:
              BUT_1=BUT_TEMP;
              FIRST_BUT=false;
            (junction 71150) -> OpCl_doors.OpCl_0.Opening0.Button_detection.BUTTON_UP.Button_UP_0 [order 1] : [PS0]
            OpCl_doors.OpCl_0.Opening0.Button_detection.BUTTON_UP.Button_UP_0 -> (junction 71151)
            (junction 71151) -> OpCl_doors.OpCl_0.Opening0.Button_detection.BUTTON_UP.First_but_0 [order 1] : [FIRST_BUT && not(RPC0)]
            OpCl_doors.OpCl_0.Opening0.Button_detection.BUTTON_UP.First_but_0 -> (junction 71152)
            (default) -> (junction 71150)
            (junction 71150) -> (junction 71155) [order 2]
            (junction 71151) -> (junction 71153) [order 2]
            (junction 71152) -> (junction 71154)
            (junction 71154) -> (junction 71153)
            (junction 71153) -> (junction 71155)
            (junction 71155) -> (junction 71156)
            (junction 71156) -> OpCl_doors.OpCl_0.Opening0.Button_detection.BUTTON_UP.Button_UP_1 [order 1] : [PS1]
            OpCl_doors.OpCl_0.Opening0.Button_detection.BUTTON_UP.Button_UP_1 -> (junction 71157)
            (junction 71157) -> OpCl_doors.OpCl_0.Opening0.Button_detection.BUTTON_UP.First_but_1 [order 1] : [FIRST_BUT && not(RPC1)]
            OpCl_doors.OpCl_0.Opening0.Button_detection.BUTTON_UP.First_but_1 -> (junction 71158)
            (junction 71156) -> (junction 71159) [order 2]
            (junction 71157) -> (junction 71160) [order 2]
            (junction 71158) -> (junction 71161)
            (junction 71160) -> (junction 71159)
            (junction 71161) -> (junction 71160)
            (junction 71159) -> (junction 71163)
            OpCl_doors.OpCl_0.Opening0.Button_detection.BUTTON_UP.First_but_2 -> (junction 71162)
            (junction 71162) -> (junction 71167)
            (junction 71163) -> OpCl_doors.OpCl_0.Opening0.Button_detection.BUTTON_UP.Button_UP_2 [order 1] : [PS2]
            OpCl_doors.OpCl_0.Opening0.Button_detection.BUTTON_UP.Button_UP_2 -> (junction 71164)
            (junction 71164) -> OpCl_doors.OpCl_0.Opening0.Button_detection.BUTTON_UP.First_but_2 [order 1] : [FIRST_BUT && not(RPC2)]
            (junction 71163) -> (junction 71165) [order 2]
            (junction 71164) -> (junction 71166) [order 2]
            (junction 71166) -> (junction 71165)
            (junction 71167) -> (junction 71166)
          state Max_Min_assignment
            state Min_but
              en:
              BUTTON=MIN_BUT;
            state Max_but
              en:
              BUTTON=MAX_BUT;
            state First_but
              en:
              BUTTON=BUT_1;
            state Max_but1
              en:
              MAX_BUT=2;
            state Max_but2
              en:
              MAX_BUT=1;
            state Max_but3
              en:
              MAX_BUT=0;
            state Min_but1
              en:
              MIN_BUT=1;
            state Min_but2
              en:
              MIN_BUT=2;
            state Min_but3
              en:
              MIN_BUT=3;
            state MAX
              en:
              MAX_BUT=BUT_TEMP;
            state MIN
              en:
              MIN_BUT=BUT_TEMP;
            state Updating_button_0
              en:
              BUTTON=MAX_BUT;
            state Updating_button_1
              en:
              BUTTON=MIN_BUT;
            (junction 71205) -> OpCl_doors.OpCl_0.Opening0.Button_detection.Max_Min_assignment.Min_but [order 1] : [(MAX_BUT-FLOOR)>(FLOOR-MIN_BUT)]
            OpCl_doors.OpCl_0.Opening0.Button_detection.Max_Min_assignment.Min_but -> (junction 71206)
            (junction 71207) -> (junction 71205) [order 1] : [not(FLAG_STOP) && MOTION==2 && FLAG==3]
            (default) -> (junction 71207)
            (junction 71205) -> (junction 71208) [order 2]
            (junction 71206) -> (junction 71209)
            (junction 71207) -> (junction 71210) [order 2]
            (junction 71208) -> OpCl_doors.OpCl_0.Opening0.Button_detection.Max_Min_assignment.Max_but [order 1] : [(MAX_BUT-FLOOR)<(FLOOR-MIN_BUT)]
            OpCl_doors.OpCl_0.Opening0.Button_detection.Max_Min_assignment.Max_but -> (junction 71209)
            (junction 71208) -> OpCl_doors.OpCl_0.Opening0.Button_detection.Max_Min_assignment.First_but [order 2]
            (junction 71209) -> (junction 71212)
            OpCl_doors.OpCl_0.Opening0.Button_detection.Max_Min_assignment.First_but -> (junction 71211)
            (junction 71211) -> (junction 71210)
            (junction 71212) -> (junction 71211)
            (junction 71210) -> (junction 71213)
            (junction 71214) -> (junction 71215) [order 1] : [MOTION==0]
                | {MOTION=1;
                | UPDATE=true;}
            (junction 71215) -> OpCl_doors.OpCl_0.Opening0.Button_detection.Max_Min_assignment.Max_but1 [order 1] : [BUTTON_UP(2)]
            OpCl_doors.OpCl_0.Opening0.Button_detection.Max_Min_assignment.Max_but1 -> (junction 71216)
            (junction 71213) -> (junction 71214) [order 1] : [BUTTON==FLOOR && EXTEND]
                | {EXTEND=false;}
            (junction 71213) -> (junction 71227) [order 2]
            (junction 71214) -> (junction 71219) [order 2]
            (junction 71215) -> (junction 71217) [order 2]
            (junction 71216) -> (junction 71218)
            (junction 71217) -> OpCl_doors.OpCl_0.Opening0.Button_detection.Max_Min_assignment.Max_but2 [order 1] : [BUTTON_UP(1)]
            OpCl_doors.OpCl_0.Opening0.Button_detection.Max_Min_assignment.Max_but2 -> (junction 71218)
            (junction 71217) -> OpCl_doors.OpCl_0.Opening0.Button_detection.Max_Min_assignment.Max_but3 [order 2]
            (junction 71218) -> (junction 71221)
            OpCl_doors.OpCl_0.Opening0.Button_detection.Max_Min_assignment.Max_but3 -> (junction 71220)
            (junction 71220) -> (junction 71219)
            (junction 71221) -> (junction 71220)
            (junction 71219) -> (junction 71222)
            (junction 71222) -> (junction 71223) [order 1] : [MOTION==1]
                | {MOTION=0;
                | UPDATE=true;}
            (junction 71223) -> OpCl_doors.OpCl_0.Opening0.Button_detection.Max_Min_assignment.Min_but1 [order 1] : [BUTTON_DOWN(1)]
            OpCl_doors.OpCl_0.Opening0.Button_detection.Max_Min_assignment.Min_but1 -> (junction 71224)
            (junction 71222) -> (junction 71228) [order 2]
            (junction 71223) -> (junction 71225) [order 2]
            (junction 71224) -> (junction 71226)
            (junction 71225) -> OpCl_doors.OpCl_0.Opening0.Button_detection.Max_Min_assignment.Min_but2 [order 1] : [BUTTON_DOWN(2)]
            OpCl_doors.OpCl_0.Opening0.Button_detection.Max_Min_assignment.Min_but2 -> (junction 71226)
            (junction 71225) -> OpCl_doors.OpCl_0.Opening0.Button_detection.Max_Min_assignment.Min_but3 [order 2]
            (junction 71226) -> (junction 71230)
            OpCl_doors.OpCl_0.Opening0.Button_detection.Max_Min_assignment.Min_but3 -> (junction 71229)
            (junction 71228) -> (junction 71227)
            (junction 71229) -> (junction 71228)
            (junction 71230) -> (junction 71229)
            (junction 71227) -> (junction 71232)
            OpCl_doors.OpCl_0.Opening0.Button_detection.Max_Min_assignment.MAX -> (junction 71231)
            (junction 71232) -> (junction 71233) [order 1] : [PUSHED]
            (junction 71233) -> (junction 71234) [order 1] : [not(BUT_TEMP==FLOOR) || not(MOTION==2)]
            (junction 71234) -> OpCl_doors.OpCl_0.Opening0.Button_detection.Max_Min_assignment.MAX [order 1] : [MAX_BUT<BUT_TEMP && not(UPDATE)]
            (junction 71231) -> (junction 71236)
            (junction 71232) -> (junction 71246) [order 2]
            (junction 71233) -> (junction 71239) [order 2]
            (junction 71234) -> (junction 71235) [order 2]
            (junction 71236) -> (junction 71235)
            (junction 71235) -> (junction 71237)
            (junction 71237) -> OpCl_doors.OpCl_0.Opening0.Button_detection.Max_Min_assignment.MIN [order 1] : [MIN_BUT>BUT_TEMP && not(UPDATE)]
            OpCl_doors.OpCl_0.Opening0.Button_detection.Max_Min_assignment.MIN -> (junction 71238)
            (junction 71237) -> (junction 71240) [order 2]
            (junction 71238) -> (junction 71241)
            (junction 71240) -> (junction 71239)
            (junction 71241) -> (junction 71240)
            (junction 71239) -> (junction 71242)
            (junction 71242) -> OpCl_doors.OpCl_0.Opening0.Button_detection.Max_Min_assignment.Updating_button_0 [order 1] : [MOTION==0]
            OpCl_doors.OpCl_0.Opening0.Button_detection.Max_Min_assignment.Updating_button_0 -> (junction 71243)
            (junction 71242) -> (junction 71244) [order 2]
            (junction 71243) -> (junction 71245)
            (junction 71244) -> OpCl_doors.OpCl_0.Opening0.Button_detection.Max_Min_assignment.Updating_button_1 [order 1] : [MOTION==1]
            OpCl_doors.OpCl_0.Opening0.Button_detection.Max_Min_assignment.Updating_button_1 -> (junction 71245)
            (junction 71244) -> (junction 71247) [order 2]
            (junction 71245) -> (junction 71248)
            (junction 71247) -> (junction 71246)
            (junction 71248) -> (junction 71247)
          state GoTo_PositionControl
            en:
            BUTTON=BUT_TEMP;
            FLAG=2;
          state Emergency
            en:
            FLAG_EMG=true;
            FLAG=4;
          state Timer_EME
            state Set_tmr
              en:
              Q_EME=true;
            state Counting
              en:
              ET_EME= ET_EME + 1;
              Q_EME=false;
            state Set
              en:
              IN_EME=true;
              PT_EME=3;
            (junction 71338) -> OpCl_doors.OpCl_0.Opening0.Button_detection.Timer_EME.Set_tmr [order 1] : [ET_EME==PT_EME]
            OpCl_doors.OpCl_0.Opening0.Button_detection.Timer_EME.Set_tmr -> (junction 71339)
            OpCl_doors.OpCl_0.Opening0.Button_detection.Timer_EME.Counting -> (junction 71338)
            (junction 71338) -> (junction 71339) [order 2]
            (default) -> OpCl_doors.OpCl_0.Opening0.Button_detection.Timer_EME.Set
            OpCl_doors.OpCl_0.Opening0.Button_detection.Timer_EME.Set -> (junction 71340)
            (junction 71340) -> OpCl_doors.OpCl_0.Opening0.Button_detection.Timer_EME.Counting [order 1] : [ET_EME<PT_EME]
            (junction 71340) -> (junction 71339) [order 2]
          state Not_Emergency
            en:
            IN_EME=false;
            ET_EME=0;
          state SwitchingOFF_LEDs
            en:
            LPD3=false;
            LPD2=false;
            LPS2=false;
            LPD1=false;
            LPS1=false;
            LPS0=false;
          (default) -> (junction 70939)
          (junction 70939) -> (junction 70940) [order 1] : [FLAG==1 && not(PUSHED)]
              | {BUTTON=FLOOR;
              | BUT_TEMP=BUTTON;
              | BUT_1=FLOOR;}
          (junction 70940) -> OpCl_doors.OpCl_0.Opening0.Button_detection.Timer_LL [order 1] : [not(FLAG_STOP)]
          OpCl_doors.OpCl_0.Opening0.Button_detection.Timer_LL -> OpCl_doors.OpCl_0.Opening0.Button_detection.Save_energy
          OpCl_doors.OpCl_0.Opening0.Button_detection.Save_energy -> (junction 70941)
          (junction 70939) -> (junction 70942) [order 2]
          (junction 70940) -> (junction 70943) [order 2]
          (junction 70941) -> (junction 70944)
          (junction 70943) -> (junction 70942)
          (junction 70944) -> (junction 70943)
          (junction 70942) -> OpCl_doors.OpCl_0.Opening0.Button_detection.BUTTON_CAR
          OpCl_doors.OpCl_0.Opening0.Button_detection.BUTTON_UP -> OpCl_doors.OpCl_0.Opening0.Button_detection.BUTTON_DOWN
          OpCl_doors.OpCl_0.Opening0.Button_detection.BUTTON_DOWN -> OpCl_doors.OpCl_0.Opening0.Button_detection.Max_Min_assignment
          OpCl_doors.OpCl_0.Opening0.Button_detection.Max_Min_assignment -> (junction 70945)
          OpCl_doors.OpCl_0.Opening0.Button_detection.BUTTON_CAR -> OpCl_doors.OpCl_0.Opening0.Button_detection.BUTTON_UP
          (junction 70945) -> (junction 70947)
          (junction 70947) -> (junction 70946)
          (junction 70946) -> (junction 70949)
          (junction 70949) -> (junction 70950) [order 1] : [FLAG==1]
          (junction 70950) -> OpCl_doors.OpCl_0.Opening0.Button_detection.GoTo_PositionControl [order 1] : [PUSHED]
          OpCl_doors.OpCl_0.Opening0.Button_detection.GoTo_PositionControl -> (junction 70948)
          (junction 70949) -> (junction 70960) [order 2]
          (junction 70950) -> (junction 70951) [order 2]
          (junction 70948) -> (junction 70952)
          (junction 70952) -> (junction 70951)
          (junction 70951) -> (junction 70954)
          OpCl_doors.OpCl_0.Opening0.Button_detection.Emergency -> (junction 70953)
          (junction 70954) -> OpCl_doors.OpCl_0.Opening0.Button_detection.Timer_EME [order 1] : [STOP]
              | {IN_LL=false; ET_LL=0;FLAG=1;}
          OpCl_doors.OpCl_0.Opening0.Button_detection.Timer_EME -> (junction 70955)
          (junction 70955) -> OpCl_doors.OpCl_0.Opening0.Button_detection.Emergency [order 1] : [Q_EME]
          (junction 70953) -> (junction 70957)
          (junction 70954) -> OpCl_doors.OpCl_0.Opening0.Button_detection.Not_Emergency [order 2]
          (junction 70955) -> (junction 70956) [order 2]
          (junction 70957) -> (junction 70956)
          (junction 70956) -> (junction 70959)
          OpCl_doors.OpCl_0.Opening0.Button_detection.Not_Emergency -> (junction 70959)
          OpCl_doors.OpCl_0.Opening0.Button_detection.SwitchingOFF_LEDs -> (junction 70958)
          (junction 70959) -> OpCl_doors.OpCl_0.Opening0.Button_detection.SwitchingOFF_LEDs [order 1] : [FLAG_STOP && FLAG==2]
          (junction 70958) -> (junction 70962)
          (junction 70959) -> (junction 70961) [order 2]
          (junction 70961) -> (junction 70960)
          (junction 70962) -> (junction 70961)
        state Button_detection1
          state Save_energy
            en:
            LL=not(Q_LL);
          state Timer_LL
            state Set_tmr
              en:
              Q_LL=true;
            state Counting
              en:
              ET_LL= ET_LL + 1;
              Q_LL=false;
            state Set
              en:
              IN_LL=true;
              PT_LL=10;
            (junction 71424) -> OpCl_doors.OpCl_0.Opening0.Button_detection1.Timer_LL.Set_tmr [order 1] : [ET_LL==PT_LL]
            OpCl_doors.OpCl_0.Opening0.Button_detection1.Timer_LL.Set_tmr -> (junction 71425)
            OpCl_doors.OpCl_0.Opening0.Button_detection1.Timer_LL.Counting -> (junction 71424)
            (junction 71424) -> (junction 71425) [order 2]
            (default) -> OpCl_doors.OpCl_0.Opening0.Button_detection1.Timer_LL.Set
            OpCl_doors.OpCl_0.Opening0.Button_detection1.Timer_LL.Set -> (junction 71426)
            (junction 71426) -> OpCl_doors.OpCl_0.Opening0.Button_detection1.Timer_LL.Counting [order 1] : [ET_LL<PT_LL]
            (junction 71426) -> (junction 71425) [order 2]
          state BUTTON_DOWN
            state Button_DOWN_1
              en:
              BUTTON_DOWN(2)=true;
              BUT_TEMP=1;
              LPD1=true;
              PUSHED=true;
              UPDATE=false;
              IN_LL=false; ET_LL=0;
            state First_but_1
              en:
              BUT_1=BUT_TEMP;
              FIRST_BUT=false;
            state Button_DOWN_2
              en:
              BUTTON_DOWN(3)=true;
              BUT_TEMP=2;
              LPD2=true;
              PUSHED=true;
              UPDATE=false;
              IN_LL=false; ET_LL=0;
            state First_but_2
              en:
              BUT_1=BUT_TEMP;
              FIRST_BUT=false;
            state Button_DOWN_3
              en:
              BUTTON_DOWN(4)=true;
              BUT_TEMP=3;
              LPD3=true;
              PUSHED=true;
              UPDATE=false;
              IN_LL=false; ET_LL=0;
            state First_but_3
              en:
              BUT_1=BUT_TEMP;
              FIRST_BUT=false;
            (default) -> (junction 71439)
            (junction 71439) -> OpCl_doors.OpCl_0.Opening0.Button_detection1.BUTTON_DOWN.Button_DOWN_1 [order 1] : [PD1]
            OpCl_doors.OpCl_0.Opening0.Button_detection1.BUTTON_DOWN.Button_DOWN_1 -> (junction 71440)
            (junction 71440) -> OpCl_doors.OpCl_0.Opening0.Button_detection1.BUTTON_DOWN.First_but_1 [order 1] : [FIRST_BUT && not(RPC1)]
            OpCl_doors.OpCl_0.Opening0.Button_detection1.BUTTON_DOWN.First_but_1 -> (junction 71441)
            (junction 71439) -> (junction 71442) [order 2]
            (junction 71440) -> (junction 71443) [order 2]
            (junction 71441) -> (junction 71444)
            (junction 71443) -> (junction 71442)
            (junction 71444) -> (junction 71443)
            (junction 71442) -> (junction 71445)
            (junction 71445) -> OpCl_doors.OpCl_0.Opening0.Button_detection1.BUTTON_DOWN.Button_DOWN_2 [order 1] : [PD2]
            OpCl_doors.OpCl_0.Opening0.Button_detection1.BUTTON_DOWN.Button_DOWN_2 -> (junction 71446)
            (junction 71446) -> OpCl_doors.OpCl_0.Opening0.Button_detection1.BUTTON_DOWN.First_but_2 [order 1] : [FIRST_BUT && not(RPC2)]
            OpCl_doors.OpCl_0.Opening0.Button_detection1.BUTTON_DOWN.First_but_2 -> (junction 71447)
            (junction 71445) -> (junction 71448) [order 2]
            (junction 71446) -> (junction 71449) [order 2]
            (junction 71447) -> (junction 71450)
            (junction 71449) -> (junction 71448)
            (junction 71450) -> (junction 71449)
            (junction 71448) -> (junction 71451)
            (junction 71451) -> OpCl_doors.OpCl_0.Opening0.Button_detection1.BUTTON_DOWN.Button_DOWN_3 [order 1] : [PD3]
            OpCl_doors.OpCl_0.Opening0.Button_detection1.BUTTON_DOWN.Button_DOWN_3 -> (junction 71452)
            (junction 71452) -> OpCl_doors.OpCl_0.Opening0.Button_detection1.BUTTON_DOWN.First_but_3 [order 1] : [FIRST_BUT && not(RPC3)]
            OpCl_doors.OpCl_0.Opening0.Button_detection1.BUTTON_DOWN.First_but_3 -> (junction 71453)
            (junction 71451) -> (junction 71454) [order 2]
            (junction 71452) -> (junction 71455) [order 2]
            (junction 71453) -> (junction 71456)
            (junction 71455) -> (junction 71454)
            (junction 71456) -> (junction 71455)
          state BUTTON_CAR
            state Button_CAR_0
              en:
              BUTTON_CAR(1)=true;
              BUT_TEMP=0;
              LPC0=true;
              PUSHED=true;
              UPDATE=false;
              IN_LL=false; ET_LL=0;
            state First_but_0
              en:
              BUT_1=BUT_TEMP;
              FIRST_BUT=false;
            state Button_CAR_1
              en:
              BUTTON_CAR(2)=true;
              BUT_TEMP=1;
              LPC1=true;
              PUSHED=true;
              UPDATE=false;
              IN_LL=false; ET_LL=0;
            state First_but_1
              en:
              BUT_1=BUT_TEMP;
              FIRST_BUT=false;
            state Button_CAR_2
              en:
              BUTTON_CAR(3)=true;
              BUT_TEMP=2;
              LPC2=true;
              PUSHED=true;
              UPDATE=false;
              IN_LL=false; ET_LL=0;
            state First_but_2
              en:
              BUT_1=BUT_TEMP;
              FIRST_BUT=false;
            state Button_CAR_3
              en:
              BUTTON_CAR(4)=true;
              BUT_TEMP=3;
              LPC3=true;
              PUSHED=true;
              UPDATE=false;
              IN_LL=false; ET_LL=0;
            state First_but_3
              en:
              BUT_1=BUT_TEMP;
              FIRST_BUT=false;
            (default) -> (junction 71494)
            (junction 71494) -> OpCl_doors.OpCl_0.Opening0.Button_detection1.BUTTON_CAR.Button_CAR_0 [order 1] : [P0]
            OpCl_doors.OpCl_0.Opening0.Button_detection1.BUTTON_CAR.Button_CAR_0 -> (junction 71495)
            (junction 71495) -> OpCl_doors.OpCl_0.Opening0.Button_detection1.BUTTON_CAR.First_but_0 [order 1] : [FIRST_BUT && not(RPC0)]
            OpCl_doors.OpCl_0.Opening0.Button_detection1.BUTTON_CAR.First_but_0 -> (junction 71496)
            (junction 71494) -> (junction 71497) [order 2]
            (junction 71495) -> (junction 71498) [order 2]
            (junction 71496) -> (junction 71499)
            (junction 71498) -> (junction 71497)
            (junction 71499) -> (junction 71498)
            (junction 71497) -> (junction 71502)
            OpCl_doors.OpCl_0.Opening0.Button_detection1.BUTTON_CAR.Button_CAR_1 -> (junction 71500)
            (junction 71500) -> OpCl_doors.OpCl_0.Opening0.Button_detection1.BUTTON_CAR.First_but_1 [order 1] : [FIRST_BUT && not(RPC1)]
            OpCl_doors.OpCl_0.Opening0.Button_detection1.BUTTON_CAR.First_but_1 -> (junction 71501)
            (junction 71500) -> (junction 71504) [order 2]
            (junction 71501) -> (junction 71505)
            (junction 71502) -> OpCl_doors.OpCl_0.Opening0.Button_detection1.BUTTON_CAR.Button_CAR_1 [order 1] : [P1]
            (junction 71502) -> (junction 71503) [order 2]
            (junction 71504) -> (junction 71503)
            (junction 71505) -> (junction 71504)
            (junction 71503) -> (junction 71506)
            (junction 71506) -> OpCl_doors.OpCl_0.Opening0.Button_detection1.BUTTON_CAR.Button_CAR_2 [order 1] : [P2]
            OpCl_doors.OpCl_0.Opening0.Button_detection1.BUTTON_CAR.Button_CAR_2 -> (junction 71507)
            (junction 71507) -> OpCl_doors.OpCl_0.Opening0.Button_detection1.BUTTON_CAR.First_but_2 [order 1] : [FIRST_BUT && not(RPC2)]
            OpCl_doors.OpCl_0.Opening0.Button_detection1.BUTTON_CAR.First_but_2 -> (junction 71508)
            (junction 71506) -> (junction 71509) [order 2]
            (junction 71507) -> (junction 71510) [order 2]
            (junction 71508) -> (junction 71511)
            (junction 71510) -> (junction 71509)
            (junction 71511) -> (junction 71510)
            (junction 71509) -> (junction 71512)
            (junction 71512) -> OpCl_doors.OpCl_0.Opening0.Button_detection1.BUTTON_CAR.Button_CAR_3 [order 1] : [P3]
            OpCl_doors.OpCl_0.Opening0.Button_detection1.BUTTON_CAR.Button_CAR_3 -> (junction 71513)
            (junction 71513) -> OpCl_doors.OpCl_0.Opening0.Button_detection1.BUTTON_CAR.First_but_3 [order 1] : [FIRST_BUT && not(RPC3)]
            OpCl_doors.OpCl_0.Opening0.Button_detection1.BUTTON_CAR.First_but_3 -> (junction 71514)
            (junction 71512) -> (junction 71515) [order 2]
            (junction 71513) -> (junction 71516) [order 2]
            (junction 71514) -> (junction 71517)
            (junction 71516) -> (junction 71515)
            (junction 71517) -> (junction 71516)
          state BUTTON_UP
            state Button_UP_0
              en:
              BUTTON_UP(1)=true;
              BUT_TEMP=0;
              LPS0=true;
              PUSHED=true;
              UPDATE=false;
              IN_LL=false; ET_LL=0;
            state First_but_0
              en:
              BUT_1=BUT_TEMP;
              FIRST_BUT=false;
            state Button_UP_1
              en:
              BUTTON_UP(2)=true;
              BUT_TEMP=1;
              LPS1=true;
              PUSHED=true;
              UPDATE=false;
              IN_LL=false; ET_LL=0;
            state First_but_1
              en:
              BUT_1=BUT_TEMP;
              FIRST_BUT=false;
            state Button_UP_2
              en:
              BUTTON_UP(3)=true;
              BUT_TEMP=2;
              LPS2=true;
              PUSHED=true;
              UPDATE=false;
              IN_LL=false; ET_LL=0;
            state First_but_2
              en:
              BUT_1=BUT_TEMP;
              FIRST_BUT=false;
            (junction 71567) -> OpCl_doors.OpCl_0.Opening0.Button_detection1.BUTTON_UP.Button_UP_0 [order 1] : [PS0]
            OpCl_doors.OpCl_0.Opening0.Button_detection1.BUTTON_UP.Button_UP_0 -> (junction 71568)
            (junction 71568) -> OpCl_doors.OpCl_0.Opening0.Button_detection1.BUTTON_UP.First_but_0 [order 1] : [FIRST_BUT && not(RPC0)]
            OpCl_doors.OpCl_0.Opening0.Button_detection1.BUTTON_UP.First_but_0 -> (junction 71569)
            (default) -> (junction 71567)
            (junction 71567) -> (junction 71572) [order 2]
            (junction 71568) -> (junction 71570) [order 2]
            (junction 71569) -> (junction 71571)
            (junction 71571) -> (junction 71570)
            (junction 71570) -> (junction 71572)
            (junction 71572) -> (junction 71573)
            (junction 71573) -> OpCl_doors.OpCl_0.Opening0.Button_detection1.BUTTON_UP.Button_UP_1 [order 1] : [PS1]
            OpCl_doors.OpCl_0.Opening0.Button_detection1.BUTTON_UP.Button_UP_1 -> (junction 71574)
            (junction 71574) -> OpCl_doors.OpCl_0.Opening0.Button_detection1.BUTTON_UP.First_but_1 [order 1] : [FIRST_BUT && not(RPC1)]
            OpCl_doors.OpCl_0.Opening0.Button_detection1.BUTTON_UP.First_but_1 -> (junction 71575)
            (junction 71573) -> (junction 71576) [order 2]
            (junction 71574) -> (junction 71577) [order 2]
            (junction 71575) -> (junction 71578)
            (junction 71577) -> (junction 71576)
            (junction 71578) -> (junction 71577)
            (junction 71576) -> (junction 71580)
            OpCl_doors.OpCl_0.Opening0.Button_detection1.BUTTON_UP.First_but_2 -> (junction 71579)
            (junction 71579) -> (junction 71584)
            (junction 71580) -> OpCl_doors.OpCl_0.Opening0.Button_detection1.BUTTON_UP.Button_UP_2 [order 1] : [PS2]
            OpCl_doors.OpCl_0.Opening0.Button_detection1.BUTTON_UP.Button_UP_2 -> (junction 71581)
            (junction 71581) -> OpCl_doors.OpCl_0.Opening0.Button_detection1.BUTTON_UP.First_but_2 [order 1] : [FIRST_BUT && not(RPC2)]
            (junction 71580) -> (junction 71582) [order 2]
            (junction 71581) -> (junction 71583) [order 2]
            (junction 71583) -> (junction 71582)
            (junction 71584) -> (junction 71583)
          state Max_Min_assignment
            state Min_but
              en:
              BUTTON=MIN_BUT;
            state Max_but
              en:
              BUTTON=MAX_BUT;
            state First_but
              en:
              BUTTON=BUT_1;
            state Max_but1
              en:
              MAX_BUT=2;
            state Max_but2
              en:
              MAX_BUT=1;
            state Max_but3
              en:
              MAX_BUT=0;
            state Min_but1
              en:
              MIN_BUT=1;
            state Min_but2
              en:
              MIN_BUT=2;
            state Min_but3
              en:
              MIN_BUT=3;
            state MAX
              en:
              MAX_BUT=BUT_TEMP;
            state MIN
              en:
              MIN_BUT=BUT_TEMP;
            state Updating_button_0
              en:
              BUTTON=MAX_BUT;
            state Updating_button_1
              en:
              BUTTON=MIN_BUT;
            (junction 71622) -> OpCl_doors.OpCl_0.Opening0.Button_detection1.Max_Min_assignment.Min_but [order 1] : [(MAX_BUT-FLOOR)>(FLOOR-MIN_BUT)]
            OpCl_doors.OpCl_0.Opening0.Button_detection1.Max_Min_assignment.Min_but -> (junction 71623)
            (junction 71624) -> (junction 71622) [order 1] : [not(FLAG_STOP) && MOTION==2 && FLAG==3]
            (default) -> (junction 71624)
            (junction 71622) -> (junction 71625) [order 2]
            (junction 71623) -> (junction 71626)
            (junction 71624) -> (junction 71627) [order 2]
            (junction 71625) -> OpCl_doors.OpCl_0.Opening0.Button_detection1.Max_Min_assignment.Max_but [order 1] : [(MAX_BUT-FLOOR)<(FLOOR-MIN_BUT)]
            OpCl_doors.OpCl_0.Opening0.Button_detection1.Max_Min_assignment.Max_but -> (junction 71626)
            (junction 71625) -> OpCl_doors.OpCl_0.Opening0.Button_detection1.Max_Min_assignment.First_but [order 2]
            (junction 71626) -> (junction 71629)
            OpCl_doors.OpCl_0.Opening0.Button_detection1.Max_Min_assignment.First_but -> (junction 71628)
            (junction 71628) -> (junction 71627)
            (junction 71629) -> (junction 71628)
            (junction 71627) -> (junction 71630)
            (junction 71631) -> (junction 71632) [order 1] : [MOTION==0]
                | {MOTION=1;
                | UPDATE=true;}
            (junction 71632) -> OpCl_doors.OpCl_0.Opening0.Button_detection1.Max_Min_assignment.Max_but1 [order 1] : [BUTTON_UP(2)]
            OpCl_doors.OpCl_0.Opening0.Button_detection1.Max_Min_assignment.Max_but1 -> (junction 71633)
            (junction 71630) -> (junction 71631) [order 1] : [BUTTON==FLOOR && EXTEND]
                | {EXTEND=false;}
            (junction 71630) -> (junction 71644) [order 2]
            (junction 71631) -> (junction 71636) [order 2]
            (junction 71632) -> (junction 71634) [order 2]
            (junction 71633) -> (junction 71635)
            (junction 71634) -> OpCl_doors.OpCl_0.Opening0.Button_detection1.Max_Min_assignment.Max_but2 [order 1] : [BUTTON_UP(1)]
            OpCl_doors.OpCl_0.Opening0.Button_detection1.Max_Min_assignment.Max_but2 -> (junction 71635)
            (junction 71634) -> OpCl_doors.OpCl_0.Opening0.Button_detection1.Max_Min_assignment.Max_but3 [order 2]
            (junction 71635) -> (junction 71638)
            OpCl_doors.OpCl_0.Opening0.Button_detection1.Max_Min_assignment.Max_but3 -> (junction 71637)
            (junction 71637) -> (junction 71636)
            (junction 71638) -> (junction 71637)
            (junction 71636) -> (junction 71639)
            (junction 71639) -> (junction 71640) [order 1] : [MOTION==1]
                | {MOTION=0;
                | UPDATE=true;}
            (junction 71640) -> OpCl_doors.OpCl_0.Opening0.Button_detection1.Max_Min_assignment.Min_but1 [order 1] : [BUTTON_DOWN(1)]
            OpCl_doors.OpCl_0.Opening0.Button_detection1.Max_Min_assignment.Min_but1 -> (junction 71641)
            (junction 71639) -> (junction 71645) [order 2]
            (junction 71640) -> (junction 71642) [order 2]
            (junction 71641) -> (junction 71643)
            (junction 71642) -> OpCl_doors.OpCl_0.Opening0.Button_detection1.Max_Min_assignment.Min_but2 [order 1] : [BUTTON_DOWN(2)]
            OpCl_doors.OpCl_0.Opening0.Button_detection1.Max_Min_assignment.Min_but2 -> (junction 71643)
            (junction 71642) -> OpCl_doors.OpCl_0.Opening0.Button_detection1.Max_Min_assignment.Min_but3 [order 2]
            (junction 71643) -> (junction 71647)
            OpCl_doors.OpCl_0.Opening0.Button_detection1.Max_Min_assignment.Min_but3 -> (junction 71646)
            (junction 71645) -> (junction 71644)
            (junction 71646) -> (junction 71645)
            (junction 71647) -> (junction 71646)
            (junction 71644) -> (junction 71649)
            OpCl_doors.OpCl_0.Opening0.Button_detection1.Max_Min_assignment.MAX -> (junction 71648)
            (junction 71649) -> (junction 71650) [order 1] : [PUSHED]
            (junction 71650) -> (junction 71651) [order 1] : [not(BUT_TEMP==FLOOR) || not(MOTION==2)]
            (junction 71651) -> OpCl_doors.OpCl_0.Opening0.Button_detection1.Max_Min_assignment.MAX [order 1] : [MAX_BUT<BUT_TEMP && not(UPDATE)]
            (junction 71648) -> (junction 71653)
            (junction 71649) -> (junction 71663) [order 2]
            (junction 71650) -> (junction 71656) [order 2]
            (junction 71651) -> (junction 71652) [order 2]
            (junction 71653) -> (junction 71652)
            (junction 71652) -> (junction 71654)
            (junction 71654) -> OpCl_doors.OpCl_0.Opening0.Button_detection1.Max_Min_assignment.MIN [order 1] : [MIN_BUT>BUT_TEMP && not(UPDATE)]
            OpCl_doors.OpCl_0.Opening0.Button_detection1.Max_Min_assignment.MIN -> (junction 71655)
            (junction 71654) -> (junction 71657) [order 2]
            (junction 71655) -> (junction 71658)
            (junction 71657) -> (junction 71656)
            (junction 71658) -> (junction 71657)
            (junction 71656) -> (junction 71659)
            (junction 71659) -> OpCl_doors.OpCl_0.Opening0.Button_detection1.Max_Min_assignment.Updating_button_0 [order 1] : [MOTION==0]
            OpCl_doors.OpCl_0.Opening0.Button_detection1.Max_Min_assignment.Updating_button_0 -> (junction 71660)
            (junction 71659) -> (junction 71661) [order 2]
            (junction 71660) -> (junction 71662)
            (junction 71661) -> OpCl_doors.OpCl_0.Opening0.Button_detection1.Max_Min_assignment.Updating_button_1 [order 1] : [MOTION==1]
            OpCl_doors.OpCl_0.Opening0.Button_detection1.Max_Min_assignment.Updating_button_1 -> (junction 71662)
            (junction 71661) -> (junction 71664) [order 2]
            (junction 71662) -> (junction 71665)
            (junction 71664) -> (junction 71663)
            (junction 71665) -> (junction 71664)
          state GoTo_PositionControl
            en:
            BUTTON=BUT_TEMP;
            FLAG=2;
          state Emergency
            en:
            FLAG_EMG=true;
            FLAG=4;
          state Timer_EME
            state Set_tmr
              en:
              Q_EME=true;
            state Counting
              en:
              ET_EME= ET_EME + 1;
              Q_EME=false;
            state Set
              en:
              IN_EME=true;
              PT_EME=3;
            (junction 71755) -> OpCl_doors.OpCl_0.Opening0.Button_detection1.Timer_EME.Set_tmr [order 1] : [ET_EME==PT_EME]
            OpCl_doors.OpCl_0.Opening0.Button_detection1.Timer_EME.Set_tmr -> (junction 71756)
            OpCl_doors.OpCl_0.Opening0.Button_detection1.Timer_EME.Counting -> (junction 71755)
            (junction 71755) -> (junction 71756) [order 2]
            (default) -> OpCl_doors.OpCl_0.Opening0.Button_detection1.Timer_EME.Set
            OpCl_doors.OpCl_0.Opening0.Button_detection1.Timer_EME.Set -> (junction 71757)
            (junction 71757) -> OpCl_doors.OpCl_0.Opening0.Button_detection1.Timer_EME.Counting [order 1] : [ET_EME<PT_EME]
            (junction 71757) -> (junction 71756) [order 2]
          state Not_Emergency
            en:
            IN_EME=false;
            ET_EME=0;
          state SwitchingOFF_LEDs
            en:
            LPD3=false;
            LPD2=false;
            LPS2=false;
            LPD1=false;
            LPS1=false;
            LPS0=false;
          (default) -> (junction 71356)
          (junction 71356) -> (junction 71357) [order 1] : [FLAG==1 && not(PUSHED)]
              | {BUTTON=FLOOR;
              | BUT_TEMP=BUTTON;
              | BUT_1=FLOOR;}
          (junction 71357) -> OpCl_doors.OpCl_0.Opening0.Button_detection1.Timer_LL [order 1] : [not(FLAG_STOP)]
          OpCl_doors.OpCl_0.Opening0.Button_detection1.Save_energy -> (junction 71358)
          OpCl_doors.OpCl_0.Opening0.Button_detection1.Timer_LL -> OpCl_doors.OpCl_0.Opening0.Button_detection1.Save_energy
          (junction 71357) -> (junction 71360) [order 2]
          (junction 71356) -> (junction 71359) [order 2]
          (junction 71358) -> (junction 71361)
          (junction 71360) -> (junction 71359)
          (junction 71361) -> (junction 71360)
          (junction 71359) -> OpCl_doors.OpCl_0.Opening0.Button_detection1.BUTTON_CAR
          OpCl_doors.OpCl_0.Opening0.Button_detection1.BUTTON_UP -> OpCl_doors.OpCl_0.Opening0.Button_detection1.BUTTON_DOWN
          OpCl_doors.OpCl_0.Opening0.Button_detection1.BUTTON_DOWN -> OpCl_doors.OpCl_0.Opening0.Button_detection1.Max_Min_assignment
          OpCl_doors.OpCl_0.Opening0.Button_detection1.Max_Min_assignment -> (junction 71362)
          OpCl_doors.OpCl_0.Opening0.Button_detection1.BUTTON_CAR -> OpCl_doors.OpCl_0.Opening0.Button_detection1.BUTTON_UP
          (junction 71362) -> (junction 71364)
          (junction 71364) -> (junction 71363)
          (junction 71363) -> (junction 71366)
          OpCl_doors.OpCl_0.Opening0.Button_detection1.GoTo_PositionControl -> (junction 71365)
          (junction 71366) -> (junction 71367) [order 1] : [FLAG==1]
          (junction 71367) -> OpCl_doors.OpCl_0.Opening0.Button_detection1.GoTo_PositionControl [order 1] : [PUSHED]
          (junction 71365) -> (junction 71369)
          (junction 71366) -> (junction 71377) [order 2]
          (junction 71367) -> (junction 71368) [order 2]
          (junction 71369) -> (junction 71368)
          (junction 71368) -> (junction 71371)
          OpCl_doors.OpCl_0.Opening0.Button_detection1.Emergency -> (junction 71370)
          (junction 71371) -> OpCl_doors.OpCl_0.Opening0.Button_detection1.Timer_EME [order 1] : [STOP]
              | {IN_LL=false; ET_LL=0;FLAG=1;}
          OpCl_doors.OpCl_0.Opening0.Button_detection1.Timer_EME -> (junction 71372)
          (junction 71372) -> OpCl_doors.OpCl_0.Opening0.Button_detection1.Emergency [order 1] : [Q_EME]
          (junction 71370) -> (junction 71374)
          (junction 71371) -> OpCl_doors.OpCl_0.Opening0.Button_detection1.Not_Emergency [order 2]
          (junction 71372) -> (junction 71373) [order 2]
          (junction 71374) -> (junction 71373)
          (junction 71373) -> (junction 71376)
          OpCl_doors.OpCl_0.Opening0.Button_detection1.Not_Emergency -> (junction 71376)
          OpCl_doors.OpCl_0.Opening0.Button_detection1.SwitchingOFF_LEDs -> (junction 71375)
          (junction 71376) -> OpCl_doors.OpCl_0.Opening0.Button_detection1.SwitchingOFF_LEDs [order 1] : [FLAG_STOP && FLAG==2]
          (junction 71375) -> (junction 71379)
          (junction 71376) -> (junction 71378) [order 2]
          (junction 71378) -> (junction 71377)
          (junction 71379) -> (junction 71378)
        state Opening1
          en:AP0=true;
        state Reset
          state Reset_0
            en:
            LPS0=false;
            BUTTON_CAR(1)=false;
            BUTTON_UP(1)=false;
          state Reset_1
            en:
            LPS1=false;
            LPD1=false;
            BUTTON_CAR(2)=false;
            BUTTON_UP(2)=false;
            BUTTON_DOWN(2)=false;
          state Reset_2
            en:
            LPS2=false;
            LPD2=false;
            BUTTON_CAR(3)=false;
            BUTTON_UP(3)=false;
            BUTTON_DOWN(3)=false;
          state Reset_3
            en:
            LPD3=false;
            BUTTON_CAR(4)=false;
            BUTTON_DOWN(4)=false;
          (default) -> (junction 80953)
          (junction 80953) -> OpCl_doors.OpCl_0.Opening0.Reset.Reset_0 [order 1] : [FLOOR==0]
          OpCl_doors.OpCl_0.Opening0.Reset.Reset_0 -> (junction 80954)
          (junction 80953) -> (junction 80955) [order 2]
          (junction 80954) -> (junction 80956)
          (junction 80955) -> OpCl_doors.OpCl_0.Opening0.Reset.Reset_1 [order 1] : [FLOOR==1]
          OpCl_doors.OpCl_0.Opening0.Reset.Reset_1 -> (junction 80956)
          (junction 80955) -> (junction 80957) [order 2]
          (junction 80956) -> (junction 80958)
          (junction 80957) -> OpCl_doors.OpCl_0.Opening0.Reset.Reset_2 [order 1] : [FLOOR==2]
          OpCl_doors.OpCl_0.Opening0.Reset.Reset_2 -> (junction 80958)
          (junction 80957) -> (junction 80959) [order 2]
          (junction 80958) -> (junction 80960)
          (junction 80959) -> OpCl_doors.OpCl_0.Opening0.Reset.Reset_3 [order 1] : [FLOOR==3]
          OpCl_doors.OpCl_0.Opening0.Reset.Reset_3 -> (junction 80960)
          (junction 80959) -> (junction 80961) [order 2]
          (junction 80960) -> (junction 80962)
          (junction 80962) -> (junction 80961)
        state Stop_Opening1
          en: AP0=false;
          FLAG_OD=true;
          IN_cl=false;
          ET_cl=0;
        (junction 80993) -> (junction 12567)
        (junction 12567) -> (junction 80935) [order 1] : [not(OBS) ]
        (junction 80935) -> (junction 80940) [order 2]
        (junction 80940) -> OpCl_doors.OpCl_0.Opening0.Timer_open
        OpCl_doors.OpCl_0.Opening0.Timer_open -> (junction 12566)
        (junction 12566) -> OpCl_doors.OpCl_0.Opening0.Opening [order 1] : [not(PA0)]
        (default) -> OpCl_doors.OpCl_0.Opening0.People_IN
        (junction 12567) -> (junction 88206) [order 2]
        (junction 80935) -> OpCl_doors.OpCl_0.Opening0.Button_detection [order 1] : [not(FLAG==4)]
        (junction 80941) -> (junction 80940)
        (junction 80988) -> (junction 80993)
        (junction 12566) -> OpCl_doors.OpCl_0.Opening0.Stop_Opening [order 2]
        OpCl_doors.OpCl_0.Opening0.People_IN -> OpCl_doors.OpCl_0.Opening0.People_OUT
        OpCl_doors.OpCl_0.Opening0.Opening -> (junction 30593)
        (junction 88206) -> (junction 88210) [order 2]
        (junction 88206) -> OpCl_doors.OpCl_0.Opening0.Button_detection1 [order 1] : [not(FLAG==4)]
        (junction 88210) -> (junction 88213)
        OpCl_doors.OpCl_0.Opening0.Button_detection -> (junction 80941)
        OpCl_doors.OpCl_0.Opening0.People_OUT -> (junction 80950)
        OpCl_doors.OpCl_0.Opening0.Button_detection1 -> (junction 88208)
        (junction 88213) -> (junction 88208)
        (junction 80950) -> (junction 80988) [order 2]
        (junction 80950) -> OpCl_doors.OpCl_0.Opening0.Reset [order 1] : [not(FLAG==4)]
        (junction 88208) -> (junction 12568)
        (junction 80989) -> (junction 80988)
        OpCl_doors.OpCl_0.Opening0.Stop_Opening -> (junction 30591)
        (junction 12568) -> OpCl_doors.OpCl_0.Opening0.Opening1 [order 1] : [not(PA0)]
        (junction 12568) -> OpCl_doors.OpCl_0.Opening0.Stop_Opening1 [order 2]
        (junction 30593) -> (junction 30591)
        (junction 30591) -> (junction 30596)
        OpCl_doors.OpCl_0.Opening0.Opening1 -> (junction 30605)
        OpCl_doors.OpCl_0.Opening0.Reset -> (junction 80986)
        OpCl_doors.OpCl_0.Opening0.Stop_Opening1 -> (junction 30605)
        (junction 30605) -> (junction 30596)
        (junction 80986) -> (junction 80989)
      (default) -> (junction 12509)
      (junction 12509) -> (junction 12508) [order 1] : [FLAG_OD]
      (junction 12508) -> OpCl_doors.OpCl_0.Closing0 [order 1] : [not(SWITCH) && not(STOP) && WEIGHT<=320 && not(PS0 || P0) ]
      OpCl_doors.OpCl_0.Closing0 -> (junction 30469)
      (junction 12509) -> OpCl_doors.OpCl_0.Opening0 [order 2]
      (junction 12508) -> OpCl_doors.OpCl_0.StopClosing [order 2]
      (junction 30469) -> (junction 30471)
      OpCl_doors.OpCl_0.StopClosing -> (junction 30467)
      (junction 30471) -> (junction 30467)
      (junction 30467) -> (junction 30474)
      OpCl_doors.OpCl_0.Opening0 -> (junction 30474)
    state Button_detection
      state Save_energy
        en:
        LL=not(Q_LL);
      state Timer_LL
        state Set_tmr
          en:
          Q_LL=true;
        state Counting
          en:
          ET_LL= ET_LL + 1;
          Q_LL=false;
        state Set
          en:
          IN_LL=true;
          PT_LL=10;
        (junction 68547) -> OpCl_doors.Button_detection.Timer_LL.Set_tmr [order 1] : [ET_LL==PT_LL]
        OpCl_doors.Button_detection.Timer_LL.Set_tmr -> (junction 68548)
        OpCl_doors.Button_detection.Timer_LL.Counting -> (junction 68547)
        (junction 68547) -> (junction 68548) [order 2]
        (default) -> OpCl_doors.Button_detection.Timer_LL.Set
        OpCl_doors.Button_detection.Timer_LL.Set -> (junction 68549)
        (junction 68549) -> OpCl_doors.Button_detection.Timer_LL.Counting [order 1] : [ET_LL<PT_LL]
        (junction 68549) -> (junction 68548) [order 2]
      state BUTTON_DOWN
        state Button_DOWN_1
          en:
          BUTTON_DOWN(2)=true;
          BUT_TEMP=1;
          LPD1=true;
          PUSHED=true;
          UPDATE=false;
          IN_LL=false; ET_LL=0;
        state First_but_1
          en:
          BUT_1=BUT_TEMP;
          FIRST_BUT=false;
        state Button_DOWN_2
          en:
          BUTTON_DOWN(3)=true;
          BUT_TEMP=2;
          LPD2=true;
          PUSHED=true;
          UPDATE=false;
          IN_LL=false; ET_LL=0;
        state First_but_2
          en:
          BUT_1=BUT_TEMP;
          FIRST_BUT=false;
        state Button_DOWN_3
          en:
          BUTTON_DOWN(4)=true;
          BUT_TEMP=3;
          LPD3=true;
          PUSHED=true;
          UPDATE=false;
          IN_LL=false; ET_LL=0;
        state First_but_3
          en:
          BUT_1=BUT_TEMP;
          FIRST_BUT=false;
        (default) -> (junction 68562)
        (junction 68562) -> OpCl_doors.Button_detection.BUTTON_DOWN.Button_DOWN_1 [order 1] : [PD1]
        OpCl_doors.Button_detection.BUTTON_DOWN.Button_DOWN_1 -> (junction 68563)
        (junction 68563) -> OpCl_doors.Button_detection.BUTTON_DOWN.First_but_1 [order 1] : [FIRST_BUT && not(RPC1)]
        OpCl_doors.Button_detection.BUTTON_DOWN.First_but_1 -> (junction 68564)
        (junction 68562) -> (junction 68565) [order 2]
        (junction 68563) -> (junction 68566) [order 2]
        (junction 68564) -> (junction 68567)
        (junction 68566) -> (junction 68565)
        (junction 68567) -> (junction 68566)
        (junction 68565) -> (junction 68568)
        (junction 68568) -> OpCl_doors.Button_detection.BUTTON_DOWN.Button_DOWN_2 [order 1] : [PD2]
        OpCl_doors.Button_detection.BUTTON_DOWN.Button_DOWN_2 -> (junction 68569)
        (junction 68569) -> OpCl_doors.Button_detection.BUTTON_DOWN.First_but_2 [order 1] : [FIRST_BUT && not(RPC2)]
        OpCl_doors.Button_detection.BUTTON_DOWN.First_but_2 -> (junction 68570)
        (junction 68568) -> (junction 68571) [order 2]
        (junction 68569) -> (junction 68572) [order 2]
        (junction 68570) -> (junction 68573)
        (junction 68572) -> (junction 68571)
        (junction 68573) -> (junction 68572)
        (junction 68571) -> (junction 68574)
        (junction 68574) -> OpCl_doors.Button_detection.BUTTON_DOWN.Button_DOWN_3 [order 1] : [PD3]
        OpCl_doors.Button_detection.BUTTON_DOWN.Button_DOWN_3 -> (junction 68575)
        (junction 68575) -> OpCl_doors.Button_detection.BUTTON_DOWN.First_but_3 [order 1] : [FIRST_BUT && not(RPC3)]
        OpCl_doors.Button_detection.BUTTON_DOWN.First_but_3 -> (junction 68576)
        (junction 68574) -> (junction 68577) [order 2]
        (junction 68575) -> (junction 68578) [order 2]
        (junction 68576) -> (junction 68579)
        (junction 68578) -> (junction 68577)
        (junction 68579) -> (junction 68578)
      state BUTTON_CAR
        state Button_CAR_0
          en:
          BUTTON_CAR(1)=true;
          BUT_TEMP=0;
          LPC0=true;
          PUSHED=true;
          UPDATE=false;
          IN_LL=false; ET_LL=0;
        state First_but_0
          en:
          BUT_1=BUT_TEMP;
          FIRST_BUT=false;
        state Button_CAR_1
          en:
          BUTTON_CAR(2)=true;
          BUT_TEMP=1;
          LPC1=true;
          PUSHED=true;
          UPDATE=false;
          IN_LL=false; ET_LL=0;
        state First_but_1
          en:
          BUT_1=BUT_TEMP;
          FIRST_BUT=false;
        state Button_CAR_2
          en:
          BUTTON_CAR(3)=true;
          BUT_TEMP=2;
          LPC2=true;
          PUSHED=true;
          UPDATE=false;
          IN_LL=false; ET_LL=0;
        state First_but_2
          en:
          BUT_1=BUT_TEMP;
          FIRST_BUT=false;
        state Button_CAR_3
          en:
          BUTTON_CAR(4)=true;
          BUT_TEMP=3;
          LPC3=true;
          PUSHED=true;
          UPDATE=false;
          IN_LL=false; ET_LL=0;
        state First_but_3
          en:
          BUT_1=BUT_TEMP;
          FIRST_BUT=false;
        (default) -> (junction 68617)
        (junction 68617) -> OpCl_doors.Button_detection.BUTTON_CAR.Button_CAR_0 [order 1] : [P0]
        OpCl_doors.Button_detection.BUTTON_CAR.Button_CAR_0 -> (junction 68618)
        (junction 68618) -> OpCl_doors.Button_detection.BUTTON_CAR.First_but_0 [order 1] : [FIRST_BUT && not(RPC0)]
        OpCl_doors.Button_detection.BUTTON_CAR.First_but_0 -> (junction 68619)
        (junction 68617) -> (junction 68620) [order 2]
        (junction 68618) -> (junction 68621) [order 2]
        (junction 68619) -> (junction 68622)
        (junction 68621) -> (junction 68620)
        (junction 68622) -> (junction 68621)
        (junction 68620) -> (junction 68625)
        OpCl_doors.Button_detection.BUTTON_CAR.Button_CAR_1 -> (junction 68623)
        (junction 68623) -> OpCl_doors.Button_detection.BUTTON_CAR.First_but_1 [order 1] : [FIRST_BUT && not(RPC1)]
        OpCl_doors.Button_detection.BUTTON_CAR.First_but_1 -> (junction 68624)
        (junction 68623) -> (junction 68627) [order 2]
        (junction 68624) -> (junction 68628)
        (junction 68625) -> OpCl_doors.Button_detection.BUTTON_CAR.Button_CAR_1 [order 1] : [P1]
        (junction 68625) -> (junction 68626) [order 2]
        (junction 68627) -> (junction 68626)
        (junction 68628) -> (junction 68627)
        (junction 68626) -> (junction 68629)
        (junction 68629) -> OpCl_doors.Button_detection.BUTTON_CAR.Button_CAR_2 [order 1] : [P2]
        OpCl_doors.Button_detection.BUTTON_CAR.Button_CAR_2 -> (junction 68630)
        (junction 68630) -> OpCl_doors.Button_detection.BUTTON_CAR.First_but_2 [order 1] : [FIRST_BUT && not(RPC2)]
        OpCl_doors.Button_detection.BUTTON_CAR.First_but_2 -> (junction 68631)
        (junction 68629) -> (junction 68632) [order 2]
        (junction 68630) -> (junction 68633) [order 2]
        (junction 68631) -> (junction 68634)
        (junction 68633) -> (junction 68632)
        (junction 68634) -> (junction 68633)
        (junction 68632) -> (junction 68635)
        (junction 68635) -> OpCl_doors.Button_detection.BUTTON_CAR.Button_CAR_3 [order 1] : [P3]
        OpCl_doors.Button_detection.BUTTON_CAR.Button_CAR_3 -> (junction 68636)
        (junction 68636) -> OpCl_doors.Button_detection.BUTTON_CAR.First_but_3 [order 1] : [FIRST_BUT && not(RPC3)]
        OpCl_doors.Button_detection.BUTTON_CAR.First_but_3 -> (junction 68637)
        (junction 68635) -> (junction 68638) [order 2]
        (junction 68636) -> (junction 68639) [order 2]
        (junction 68637) -> (junction 68640)
        (junction 68639) -> (junction 68638)
        (junction 68640) -> (junction 68639)
      state BUTTON_UP
        state Button_UP_0
          en:
          BUTTON_UP(1)=true;
          BUT_TEMP=0;
          LPS0=true;
          PUSHED=true;
          UPDATE=false;
          IN_LL=false; ET_LL=0;
        state First_but_0
          en:
          BUT_1=BUT_TEMP;
          FIRST_BUT=false;
        state Button_UP_1
          en:
          BUTTON_UP(2)=true;
          BUT_TEMP=1;
          LPS1=true;
          PUSHED=true;
          UPDATE=false;
          IN_LL=false; ET_LL=0;
        state First_but_1
          en:
          BUT_1=BUT_TEMP;
          FIRST_BUT=false;
        state Button_UP_2
          en:
          BUTTON_UP(3)=true;
          BUT_TEMP=2;
          LPS2=true;
          PUSHED=true;
          UPDATE=false;
          IN_LL=false; ET_LL=0;
        state First_but_2
          en:
          BUT_1=BUT_TEMP;
          FIRST_BUT=false;
        (junction 68690) -> OpCl_doors.Button_detection.BUTTON_UP.Button_UP_0 [order 1] : [PS0]
        OpCl_doors.Button_detection.BUTTON_UP.Button_UP_0 -> (junction 68691)
        (junction 68691) -> OpCl_doors.Button_detection.BUTTON_UP.First_but_0 [order 1] : [FIRST_BUT && not(RPC0)]
        OpCl_doors.Button_detection.BUTTON_UP.First_but_0 -> (junction 68692)
        (default) -> (junction 68690)
        (junction 68690) -> (junction 68695) [order 2]
        (junction 68691) -> (junction 68693) [order 2]
        (junction 68692) -> (junction 68694)
        (junction 68694) -> (junction 68693)
        (junction 68693) -> (junction 68695)
        (junction 68695) -> (junction 68696)
        (junction 68696) -> OpCl_doors.Button_detection.BUTTON_UP.Button_UP_1 [order 1] : [PS1]
        OpCl_doors.Button_detection.BUTTON_UP.Button_UP_1 -> (junction 68697)
        (junction 68697) -> OpCl_doors.Button_detection.BUTTON_UP.First_but_1 [order 1] : [FIRST_BUT && not(RPC1)]
        OpCl_doors.Button_detection.BUTTON_UP.First_but_1 -> (junction 68698)
        (junction 68696) -> (junction 68699) [order 2]
        (junction 68697) -> (junction 68700) [order 2]
        (junction 68698) -> (junction 68701)
        (junction 68700) -> (junction 68699)
        (junction 68701) -> (junction 68700)
        (junction 68699) -> (junction 68703)
        OpCl_doors.Button_detection.BUTTON_UP.First_but_2 -> (junction 68702)
        (junction 68702) -> (junction 68707)
        (junction 68703) -> OpCl_doors.Button_detection.BUTTON_UP.Button_UP_2 [order 1] : [PS2]
        OpCl_doors.Button_detection.BUTTON_UP.Button_UP_2 -> (junction 68704)
        (junction 68704) -> OpCl_doors.Button_detection.BUTTON_UP.First_but_2 [order 1] : [FIRST_BUT && not(RPC2)]
        (junction 68703) -> (junction 68705) [order 2]
        (junction 68704) -> (junction 68706) [order 2]
        (junction 68706) -> (junction 68705)
        (junction 68707) -> (junction 68706)
      state Max_Min_assignment
        state Min_but
          en:
          BUTTON=MIN_BUT;
        state Max_but
          en:
          BUTTON=MAX_BUT;
        state First_but
          en:
          BUTTON=BUT_1;
        state Max_but1
          en:
          MAX_BUT=2;
        state Max_but2
          en:
          MAX_BUT=1;
        state Max_but3
          en:
          MAX_BUT=0;
        state Min_but1
          en:
          MIN_BUT=1;
        state Min_but2
          en:
          MIN_BUT=2;
        state Min_but3
          en:
          MIN_BUT=3;
        state MAX
          en:
          MAX_BUT=BUT_TEMP;
        state MIN
          en:
          MIN_BUT=BUT_TEMP;
        state Updating_button_0
          en:
          BUTTON=MAX_BUT;
        state Updating_button_1
          en:
          BUTTON=MIN_BUT;
        (junction 68745) -> OpCl_doors.Button_detection.Max_Min_assignment.Min_but [order 1] : [(MAX_BUT-FLOOR)>(FLOOR-MIN_BUT)]
        OpCl_doors.Button_detection.Max_Min_assignment.Min_but -> (junction 68746)
        (junction 68747) -> (junction 68745) [order 1] : [not(FLAG_STOP) && MOTION==2 && FLAG==3]
        (default) -> (junction 68747)
        (junction 68745) -> (junction 68748) [order 2]
        (junction 68746) -> (junction 68749)
        (junction 68747) -> (junction 68750) [order 2]
        (junction 68748) -> OpCl_doors.Button_detection.Max_Min_assignment.Max_but [order 1] : [(MAX_BUT-FLOOR)<(FLOOR-MIN_BUT)]
        OpCl_doors.Button_detection.Max_Min_assignment.Max_but -> (junction 68749)
        (junction 68748) -> OpCl_doors.Button_detection.Max_Min_assignment.First_but [order 2]
        (junction 68749) -> (junction 68752)
        OpCl_doors.Button_detection.Max_Min_assignment.First_but -> (junction 68751)
        (junction 68751) -> (junction 68750)
        (junction 68752) -> (junction 68751)
        (junction 68750) -> (junction 68753)
        (junction 68754) -> (junction 68755) [order 1] : [MOTION==0]
            | {MOTION=1;
            | UPDATE=true;}
        (junction 68755) -> OpCl_doors.Button_detection.Max_Min_assignment.Max_but1 [order 1] : [BUTTON_UP(2)]
        OpCl_doors.Button_detection.Max_Min_assignment.Max_but1 -> (junction 68756)
        (junction 68753) -> (junction 68754) [order 1] : [BUTTON==FLOOR && EXTEND]
            | {EXTEND=false;}
        (junction 68753) -> (junction 68767) [order 2]
        (junction 68754) -> (junction 68759) [order 2]
        (junction 68755) -> (junction 68757) [order 2]
        (junction 68756) -> (junction 68758)
        (junction 68757) -> OpCl_doors.Button_detection.Max_Min_assignment.Max_but2 [order 1] : [BUTTON_UP(1)]
        OpCl_doors.Button_detection.Max_Min_assignment.Max_but2 -> (junction 68758)
        (junction 68757) -> OpCl_doors.Button_detection.Max_Min_assignment.Max_but3 [order 2]
        (junction 68758) -> (junction 68761)
        OpCl_doors.Button_detection.Max_Min_assignment.Max_but3 -> (junction 68760)
        (junction 68760) -> (junction 68759)
        (junction 68761) -> (junction 68760)
        (junction 68759) -> (junction 68762)
        (junction 68762) -> (junction 68763) [order 1] : [MOTION==1]
            | {MOTION=0;
            | UPDATE=true;}
        (junction 68763) -> OpCl_doors.Button_detection.Max_Min_assignment.Min_but1 [order 1] : [BUTTON_DOWN(1)]
        OpCl_doors.Button_detection.Max_Min_assignment.Min_but1 -> (junction 68764)
        (junction 68762) -> (junction 68768) [order 2]
        (junction 68763) -> (junction 68765) [order 2]
        (junction 68764) -> (junction 68766)
        (junction 68765) -> OpCl_doors.Button_detection.Max_Min_assignment.Min_but2 [order 1] : [BUTTON_DOWN(2)]
        OpCl_doors.Button_detection.Max_Min_assignment.Min_but2 -> (junction 68766)
        (junction 68765) -> OpCl_doors.Button_detection.Max_Min_assignment.Min_but3 [order 2]
        (junction 68766) -> (junction 68770)
        OpCl_doors.Button_detection.Max_Min_assignment.Min_but3 -> (junction 68769)
        (junction 68768) -> (junction 68767)
        (junction 68769) -> (junction 68768)
        (junction 68770) -> (junction 68769)
        (junction 68767) -> (junction 68772)
        OpCl_doors.Button_detection.Max_Min_assignment.MAX -> (junction 68771)
        (junction 68772) -> (junction 68773) [order 1] : [PUSHED]
        (junction 68773) -> (junction 68774) [order 1] : [not(BUT_TEMP==FLOOR) || not(MOTION==2)]
        (junction 68774) -> OpCl_doors.Button_detection.Max_Min_assignment.MAX [order 1] : [MAX_BUT<BUT_TEMP && not(UPDATE)]
        (junction 68771) -> (junction 68776)
